simulink library "Ta_Library"  (R2019b)
settings: Solver=VariableStepAuto  StartTime=0.0  StopTime=10.0  RelTol=1e-3
undefined symbols (not defined in the file): AEBSFunctionLib, StateDelayAbortion, TargetClassification
libraries: Mylibrary x5, simulink x1
(part 2 of 3)

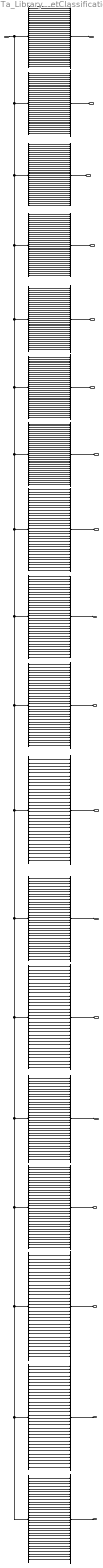
== system Ta_Library/TargetClassification ==
  Spi_input_Bus : Inport  OutDataTypeStr=Bus: Spi_input_Bus
  Bus Selector : BusSelector  OutputSignals=CAM_TGT_01A_CAN_Tgt_01_ID,CAM_TGT_02A_CAN_Tgt_02_ID,CAM_TGT_03A_CAN_Tgt_03_ID,CAM_TGT_04A_CAN_Tgt_04_ID,CAM_TGT_05A_CAN_Tgt_05_ID,CAM_TGT_06A_CAN_Tgt_06_ID,CAM_TGT_07A_CAN_Tgt_07_ID,CAM_TGT_08A_CAN_Tgt_08_ID,CAM_TGT_09A_CAN_Tgt_09_ID,CAM_TGT_10A_CAN_Tgt_10_ID,CAM_TGT_11A_CAN_Tgt_11_ID,CAM_TGT_12A_CAN_Tgt_12_ID,CAM_TGT_13A_CAN_Tgt_13_ID,CAM_TGT_14A_CAN_Tgt_14_ID,CAM_TGT_15A_CAN_Tgt_15_ID,CAM_TGT_16A_CAN_Tgt_16_ID,CAM_TGT_17A_CAN_Tgt_17_ID,CAM_TGT_18A_CAN_Tgt_18_ID,CAM_TGT_19A_CAN_Tgt_19_ID,CAM_TGT_20A_CAN_Tgt_20_ID,CAM_TGT_21A_CAN_Tgt_21_ID,CAM_TGT_22A_CAN_Tgt_22_ID,CAM_TGT_23A_CAN_Tgt_23_ID,CAM_TGT_24A_CAN_Tgt_24_ID,CAM_TGT_25A_CAN_Tgt_25_ID,CAM_TGT_26A_CAN_Tgt_26_ID,CAM_TGT_27A_CAN_Tgt_27_ID,CAM_TGT_28A_CAN_Tgt_28_ID,CAM_TGT_29A_CAN_Tgt_29_ID,CAM_TGT_30A_CAN_Tgt_30_ID,CAM_TGT_31A_CAN_Tgt_31_ID,CAM_TGT_32A_CAN_Tgt_32_ID
  Bus Selector1 : BusSelector  OutputSignals=CAM_TGT_01A_CAN_Tgt_01_Pos_Y_Quality,CAM_TGT_02A_CAN_Tgt_02_Pos_Y_Quality,CAM_TGT_03A_CAN_Tgt_03_Pos_Y_Quality,CAM_TGT_04A_CAN_Tgt_04_Pos_Y_Quality,CAM_TGT_05A_CAN_Tgt_05_Pos_Y_Quality,CAM_TGT_06A_CAN_Tgt_06_Pos_Y_Quality,CAM_TGT_07A_CAN_Tgt_07_Pos_Y_Quality,CAM_TGT_08A_CAN_Tgt_08_Pos_Y_Quality,CAM_TGT_09A_CAN_Tgt_09_Pos_Y_Quality,CAM_TGT_10A_CAN_Tgt_10_Pos_Y_Quality,CAM_TGT_11A_CAN_Tgt_11_Pos_Y_Quality,CAM_TGT_12A_CAN_Tgt_12_Pos_Y_Quality,CAM_TGT_13A_CAN_Tgt_13_Pos_Y_Quality,CAM_TGT_14A_CAN_Tgt_14_Pos_Y_Quality,CAM_TGT_15A_CAN_Tgt_15_Pos_Y_Quality,CAM_TGT_16A_CAN_Tgt_16_Pos_Y_Quality,CAM_TGT_17A_CAN_Tgt_17_Pos_Y_Quality,CAM_TGT_18A_CAN_Tgt_18_Pos_Y_Quality,CAM_TGT_19A_CAN_Tgt_19_Pos_Y_Quality,CAM_TGT_20A_CAN_Tgt_20_Pos_Y_Quality,CAM_TGT_21A_CAN_Tgt_21_Pos_Y_Quality,CAM_TGT_22A_CAN_Tgt_22_Pos_Y_Quality,CAM_TGT_23A_CAN_Tgt_23_Pos_Y_Quality,CAM_TGT_24A_CAN_Tgt_24_Pos_Y_Quality,CAM_TGT_25A_CAN_Tgt_25_Pos_Y_Quality,CAM_TGT_26A_CAN_Tgt_26_Pos_Y_Quality,CAM_TGT_27A_CAN_Tgt_27_Pos_Y_Quality,CAM_TGT_28A_CAN_Tgt_28_Pos_Y_Quality,CAM_TGT_29A_CAN_Tgt_29_Pos_Y_Quality,CAM_TGT_30A_CAN_Tgt_30_Pos_Y_Quality,CAM_TGT_31A_CAN_Tgt_31_Pos_Y_Quality,CAM_TGT_32A_CAN_Tgt_32_Pos_Y_Quality
  Bus Selector10 : BusSelector  OutputSignals=CAM_TGT_01A_CAN_Tgt_01_Pos_Y,CAM_TGT_02A_CAN_Tgt_02_Pos_Y,CAM_TGT_03A_CAN_Tgt_03_Pos_Y,CAM_TGT_04A_CAN_Tgt_04_Pos_Y,CAM_TGT_05A_CAN_Tgt_05_Pos_Y,CAM_TGT_06A_CAN_Tgt_06_Pos_Y,CAM_TGT_07A_CAN_Tgt_07_Pos_Y,CAM_TGT_08A_CAN_Tgt_08_Pos_Y,CAM_TGT_09A_CAN_Tgt_09_Pos_Y,CAM_TGT_10A_CAN_Tgt_10_Pos_Y,CAM_TGT_11A_CAN_Tgt_11_Pos_Y,CAM_TGT_12A_CAN_Tgt_12_Pos_Y,CAM_TGT_13A_CAN_Tgt_13_Pos_Y,CAM_TGT_14A_CAN_Tgt_14_Pos_Y,CAM_TGT_15A_CAN_Tgt_15_Pos_Y,CAM_TGT_16A_CAN_Tgt_16_Pos_Y,CAM_TGT_17A_CAN_Tgt_17_Pos_Y,CAM_TGT_18A_CAN_Tgt_18_Pos_Y,CAM_TGT_19A_CAN_Tgt_19_Pos_Y,CAM_TGT_20A_CAN_Tgt_20_Pos_Y,CAM_TGT_21A_CAN_Tgt_21_Pos_Y,CAM_TGT_22A_CAN_Tgt_22_Pos_Y,CAM_TGT_23A_CAN_Tgt_23_Pos_Y,CAM_TGT_24A_CAN_Tgt_24_Pos_Y,CAM_TGT_25A_CAN_Tgt_25_Pos_Y,CAM_TGT_26A_CAN_Tgt_26_Pos_Y,CAM_TGT_27A_CAN_Tgt_27_Pos_Y,CAM_TGT_28A_CAN_Tgt_28_Pos_Y,CAM_TGT_29A_CAN_Tgt_29_Pos_Y,CAM_TGT_30A_CAN_Tgt_30_Pos_Y,CAM_TGT_31A_CAN_Tgt_31_Pos_Y,CAM_TGT_32A_CAN_Tgt_32_Pos_Y
  Bus Selector11 : BusSelector  OutputSignals=CAM_TGT_01A_CAN_Tgt_01_Pos_X,CAM_TGT_02A_CAN_Tgt_02_Pos_X,CAM_TGT_03A_CAN_Tgt_03_Pos_X,CAM_TGT_04A_CAN_Tgt_04_Pos_X,CAM_TGT_05A_CAN_Tgt_05_Pos_X,CAM_TGT_06A_CAN_Tgt_06_Pos_X,CAM_TGT_07A_CAN_Tgt_07_Pos_X,CAM_TGT_08A_CAN_Tgt_08_Pos_X,CAM_TGT_09A_CAN_Tgt_09_Pos_X,CAM_TGT_10A_CAN_Tgt_10_Pos_X,CAM_TGT_11A_CAN_Tgt_11_Pos_X,CAM_TGT_12A_CAN_Tgt_12_Pos_X,CAM_TGT_13A_CAN_Tgt_13_Pos_X,CAM_TGT_14A_CAN_Tgt_14_Pos_X,CAM_TGT_15A_CAN_Tgt_15_Pos_X,CAM_TGT_16A_CAN_Tgt_16_Pos_X,CAM_TGT_17A_CAN_Tgt_17_Pos_X,CAM_TGT_18A_CAN_Tgt_18_Pos_X,CAM_TGT_19A_CAN_Tgt_19_Pos_X,CAM_TGT_20A_CAN_Tgt_20_Pos_X,CAM_TGT_21A_CAN_Tgt_21_Pos_X,CAM_TGT_22A_CAN_Tgt_22_Pos_X,CAM_TGT_23A_CAN_Tgt_23_Pos_X,CAM_TGT_24A_CAN_Tgt_24_Pos_X,CAM_TGT_25A_CAN_Tgt_25_Pos_X,CAM_TGT_26A_CAN_Tgt_26_Pos_X,CAM_TGT_27A_CAN_Tgt_27_Pos_X,CAM_TGT_28A_CAN_Tgt_28_Pos_X,CAM_TGT_29A_CAN_Tgt_29_Pos_X,CAM_TGT_30A_CAN_Tgt_30_Pos_X,CAM_TGT_31A_CAN_Tgt_31_Pos_X,CAM_TGT_32A_CAN_Tgt_32_Pos_X
  Bus Selector12 : BusSelector  OutputSignals=CAM_TGT_01B_CAN_Tgt_01_Quality,CAM_TGT_02B_CAN_Tgt_02_Quality,CAM_TGT_03B_CAN_Tgt_03_Quality,CAM_TGT_04B_CAN_Tgt_04_Quality,CAM_TGT_05B_CAN_Tgt_05_Quality,CAM_TGT_06B_CAN_Tgt_06_Quality,CAM_TGT_07B_CAN_Tgt_07_Quality,CAM_TGT_08B_CAN_Tgt_08_Quality,CAM_TGT_09B_CAN_Tgt_09_Quality,CAM_TGT_10B_CAN_Tgt_10_Quality,CAM_TGT_11B_CAN_Tgt_11_Quality,CAM_TGT_12B_CAN_Tgt_12_Quality,CAM_TGT_13B_CAN_Tgt_13_Quality,CAM_TGT_14B_CAN_Tgt_14_Quality,CAM_TGT_15B_CAN_Tgt_15_Quality,CAM_TGT_16B_CAN_Tgt_16_Quality,CAM_TGT_17B_CAN_Tgt_17_Quality,CAM_TGT_18B_CAN_Tgt_18_Quality,CAM_TGT_19B_CAN_Tgt_19_Quality,CAM_TGT_20B_CAN_Tgt_20_Quality,CAM_TGT_21B_CAN_Tgt_21_Quality,CAM_TGT_22B_CAN_Tgt_22_Quality,CAM_TGT_23B_CAN_Tgt_23_Quality,CAM_TGT_24B_CAN_Tgt_24_Quality,CAM_TGT_25B_CAN_Tgt_25_Quality,CAM_TGT_26B_CAN_Tgt_26_Quality,CAM_TGT_27B_CAN_Tgt_27_Quality,CAM_TGT_28B_CAN_Tgt_28_Quality,CAM_TGT_29B_CAN_Tgt_29_Quality,CAM_TGT_30B_CAN_Tgt_30_Quality,CAM_TGT_31B_CAN_Tgt_31_Quality,CAM_TGT_32B_CAN_Tgt_32_Quality
  Bus Selector13 : BusSelector  OutputSignals=CAM_TGT_01B_CAN_Tgt_01_Length,CAM_TGT_02B_CAN_Tgt_02_Length,CAM_TGT_03B_CAN_Tgt_03_Length,CAM_TGT_04B_CAN_Tgt_04_Length,CAM_TGT_05B_CAN_Tgt_05_Length,CAM_TGT_06B_CAN_Tgt_06_Length,CAM_TGT_07B_CAN_Tgt_07_Length,CAM_TGT_08B_CAN_Tgt_08_Length,CAM_TGT_09B_CAN_Tgt_09_Length,CAM_TGT_10B_CAN_Tgt_10_Length,CAM_TGT_11B_CAN_Tgt_11_Length,CAM_TGT_12B_CAN_Tgt_12_Length,CAM_TGT_13B_CAN_Tgt_13_Length,CAM_TGT_14B_CAN_Tgt_14_Length,CAM_TGT_15B_CAN_Tgt_15_Length,CAM_TGT_16B_CAN_Tgt_16_Length,CAM_TGT_17B_CAN_Tgt_17_Length,CAM_TGT_18B_CAN_Tgt_18_Length,CAM_TGT_19B_CAN_Tgt_19_Length,CAM_TGT_20B_CAN_Tgt_20_Length,CAM_TGT_21B_CAN_Tgt_21_Length,CAM_TGT_22B_CAN_Tgt_22_Length,CAM_TGT_23B_CAN_Tgt_23_Length,CAM_TGT_24B_CAN_Tgt_24_Length,CAM_TGT_25B_CAN_Tgt_25_Length,CAM_TGT_26B_CAN_Tgt_26_Length,CAM_TGT_27B_CAN_Tgt_27_Length,CAM_TGT_28B_CAN_Tgt_28_Length,CAM_TGT_29B_CAN_Tgt_29_Length,CAM_TGT_30B_CAN_Tgt_30_Length,CAM_TGT_31B_CAN_Tgt_31_Length,CAM_TGT_32B_CAN_Tgt_32_Length
  Bus Selector14 : BusSelector  OutputSignals=CAM_TGT_01B_CAN_Tgt_01_Time,CAM_TGT_02B_CAN_Tgt_02_Time,CAM_TGT_03B_CAN_Tgt_03_Time,CAM_TGT_04B_CAN_Tgt_04_Time,CAM_TGT_05B_CAN_Tgt_05_Time,CAM_TGT_06B_CAN_Tgt_06_Time,CAM_TGT_07B_CAN_Tgt_07_Time,CAM_TGT_08B_CAN_Tgt_08_Time,CAM_TGT_09B_CAN_Tgt_09_Time,CAM_TGT_10B_CAN_Tgt_10_Time,CAM_TGT_11B_CAN_Tgt_11_Time,CAM_TGT_12B_CAN_Tgt_12_Time,CAM_TGT_13B_CAN_Tgt_13_Time,CAM_TGT_14B_CAN_Tgt_14_Time,CAM_TGT_15B_CAN_Tgt_15_Time,CAM_TGT_16B_CAN_Tgt_16_Time,CAM_TGT_17B_CAN_Tgt_17_Time,CAM_TGT_18B_CAN_Tgt_18_Time,CAM_TGT_19B_CAN_Tgt_19_Time,CAM_TGT_20B_CAN_Tgt_20_Time,CAM_TGT_21B_CAN_Tgt_21_Time,CAM_TGT_22B_CAN_Tgt_22_Time,CAM_TGT_23B_CAN_Tgt_23_Time,CAM_TGT_24B_CAN_Tgt_24_Time,CAM_TGT_25B_CAN_Tgt_25_Time,CAM_TGT_26B_CAN_Tgt_26_Time,CAM_TGT_27B_CAN_Tgt_27_Time,CAM_TGT_28B_CAN_Tgt_28_Time,CAM_TGT_29B_CAN_Tgt_29_Time,CAM_TGT_30B_CAN_Tgt_30_Time,CAM_TGT_31B_CAN_Tgt_31_Time,CAM_TGT_32B_CAN_Tgt_32_Time
  Bus Selector15 : BusSelector  OutputSignals=CAM_TGT_01B_CAN_Tgt_01_Accel,CAM_TGT_02B_CAN_Tgt_02_Accel,CAM_TGT_03B_CAN_Tgt_03_Accel,CAM_TGT_04B_CAN_Tgt_04_Accel,CAM_TGT_05B_CAN_Tgt_05_Accel,CAM_TGT_06B_CAN_Tgt_06_Accel,CAM_TGT_07B_CAN_Tgt_07_Accel,CAM_TGT_08B_CAN_Tgt_08_Accel,CAM_TGT_09B_CAN_Tgt_09_Accel,CAM_TGT_10B_CAN_Tgt_10_Accel,CAM_TGT_11B_CAN_Tgt_11_Accel,CAM_TGT_12B_CAN_Tgt_12_Accel,CAM_TGT_13B_CAN_Tgt_13_Accel,CAM_TGT_14B_CAN_Tgt_14_Accel,CAM_TGT_15B_CAN_Tgt_15_Accel,CAM_TGT_16B_CAN_Tgt_16_Accel,CAM_TGT_17B_CAN_Tgt_17_Accel,CAM_TGT_18B_CAN_Tgt_18_Accel,CAM_TGT_19B_CAN_Tgt_19_Accel,CAM_TGT_20B_CAN_Tgt_20_Accel,CAM_TGT_21B_CAN_Tgt_21_Accel,CAM_TGT_22B_CAN_Tgt_22_Accel,CAM_TGT_23B_CAN_Tgt_23_Accel,CAM_TGT_24B_CAN_Tgt_24_Accel,CAM_TGT_25B_CAN_Tgt_25_Accel,CAM_TGT_26B_CAN_Tgt_26_Accel,CAM_TGT_27B_CAN_Tgt_27_Accel,CAM_TGT_28B_CAN_Tgt_28_Accel,CAM_TGT_29B_CAN_Tgt_29_Accel,CAM_TGT_30B_CAN_Tgt_30_Accel,CAM_TGT_31B_CAN_Tgt_31_Accel,CAM_TGT_32B_CAN_Tgt_32_Accel
  Bus Selector16 : BusSelector  OutputSignals=CAM_TGT_01B_CAN_Tgt_01_Ttc,CAM_TGT_02B_CAN_Tgt_02_Ttc,CAM_TGT_03B_CAN_Tgt_03_Ttc,CAM_TGT_04B_CAN_Tgt_04_Ttc,CAM_TGT_05B_CAN_Tgt_05_Ttc,CAM_TGT_06B_CAN_Tgt_06_Ttc,CAM_TGT_07B_CAN_Tgt_07_Ttc,CAM_TGT_08B_CAN_Tgt_08_Ttc,CAM_TGT_09B_CAN_Tgt_09_Ttc,CAM_TGT_10B_CAN_Tgt_10_Ttc,CAM_TGT_11B_CAN_Tgt_11_Ttc,CAM_TGT_12B_CAN_Tgt_12_Ttc,CAM_TGT_13B_CAN_Tgt_13_Ttc,CAM_TGT_14B_CAN_Tgt_14_Ttc,CAM_TGT_15B_CAN_Tgt_15_Ttc,CAM_TGT_16B_CAN_Tgt_16_Ttc,CAM_TGT_17B_CAN_Tgt_17_Ttc,CAM_TGT_18B_CAN_Tgt_18_Ttc,CAM_TGT_19B_CAN_Tgt_19_Ttc,CAM_TGT_20B_CAN_Tgt_20_Ttc,CAM_TGT_21B_CAN_Tgt_21_Ttc,CAM_TGT_22B_CAN_Tgt_22_Ttc,CAM_TGT_23B_CAN_Tgt_23_Ttc,CAM_TGT_24B_CAN_Tgt_24_Ttc,CAM_TGT_25B_CAN_Tgt_25_Ttc,CAM_TGT_26B_CAN_Tgt_26_Ttc,CAM_TGT_27B_CAN_Tgt_27_Ttc,CAM_TGT_28B_CAN_Tgt_28_Ttc,CAM_TGT_29B_CAN_Tgt_29_Ttc,CAM_TGT_30B_CAN_Tgt_30_Ttc,CAM_TGT_31B_CAN_Tgt_31_Ttc,CAM_TGT_32B_CAN_Tgt_32_Ttc
  Bus Selector17 : BusSelector  OutputSignals=CAM_TGT_01B_CAN_Tgt_01_Width,CAM_TGT_02B_CAN_Tgt_02_Width,CAM_TGT_03B_CAN_Tgt_03_Width,CAM_TGT_04B_CAN_Tgt_04_Width,CAM_TGT_05B_CAN_Tgt_05_Width,CAM_TGT_06B_CAN_Tgt_06_Width,CAM_TGT_07B_CAN_Tgt_07_Width,CAM_TGT_08B_CAN_Tgt_08_Width,CAM_TGT_09B_CAN_Tgt_09_Width,CAM_TGT_10B_CAN_Tgt_10_Width,CAM_TGT_11B_CAN_Tgt_11_Width,CAM_TGT_12B_CAN_Tgt_12_Width,CAM_TGT_13B_CAN_Tgt_13_Width,CAM_TGT_14B_CAN_Tgt_14_Width,CAM_TGT_15B_CAN_Tgt_15_Width,CAM_TGT_16B_CAN_Tgt_16_Width,CAM_TGT_17B_CAN_Tgt_17_Width,CAM_TGT_18B_CAN_Tgt_18_Width,CAM_TGT_19B_CAN_Tgt_19_Width,CAM_TGT_20B_CAN_Tgt_20_Width,CAM_TGT_21B_CAN_Tgt_21_Width,CAM_TGT_22B_CAN_Tgt_22_Width,CAM_TGT_23B_CAN_Tgt_23_Width,CAM_TGT_24B_CAN_Tgt_24_Width,CAM_TGT_25B_CAN_Tgt_25_Width,CAM_TGT_26B_CAN_Tgt_26_Width,CAM_TGT_27B_CAN_Tgt_27_Width,CAM_TGT_28B_CAN_Tgt_28_Width,CAM_TGT_29B_CAN_Tgt_29_Width,CAM_TGT_30B_CAN_Tgt_30_Width,CAM_TGT_31B_CAN_Tgt_31_Width,CAM_TGT_32B_CAN_Tgt_32_Width
  Bus Selector2 : BusSelector  OutputSignals=CAM_TGT_01A_CAN_Tgt_01_Type,CAM_TGT_02A_CAN_Tgt_02_Type,CAM_TGT_03A_CAN_Tgt_03_Type,CAM_TGT_04A_CAN_Tgt_04_Type,CAM_TGT_05A_CAN_Tgt_05_Type,CAM_TGT_06A_CAN_Tgt_06_Type,CAM_TGT_07A_CAN_Tgt_07_Type,CAM_TGT_08A_CAN_Tgt_08_Type,CAM_TGT_09A_CAN_Tgt_09_Type,CAM_TGT_10A_CAN_Tgt_10_Type,CAM_TGT_11A_CAN_Tgt_11_Type,CAM_TGT_12A_CAN_Tgt_12_Type,CAM_TGT_13A_CAN_Tgt_13_Type,CAM_TGT_14A_CAN_Tgt_14_Type,CAM_TGT_15A_CAN_Tgt_15_Type,CAM_TGT_16A_CAN_Tgt_16_Type,CAM_TGT_17A_CAN_Tgt_17_Type,CAM_TGT_18A_CAN_Tgt_18_Type,CAM_TGT_19A_CAN_Tgt_19_Type,CAM_TGT_20A_CAN_Tgt_20_Type,CAM_TGT_21A_CAN_Tgt_21_Type,CAM_TGT_22A_CAN_Tgt_22_Type,CAM_TGT_23A_CAN_Tgt_23_Type,CAM_TGT_24A_CAN_Tgt_24_Type,CAM_TGT_25A_CAN_Tgt_25_Type,CAM_TGT_26A_CAN_Tgt_26_Type,CAM_TGT_27A_CAN_Tgt_27_Type,CAM_TGT_28A_CAN_Tgt_28_Type,CAM_TGT_29A_CAN_Tgt_29_Type,CAM_TGT_30A_CAN_Tgt_30_Type,CAM_TGT_31A_CAN_Tgt_31_Type,CAM_TGT_32A_CAN_Tgt_32_Type
  Bus Selector3 : BusSelector  OutputSignals=CAM_TGT_01A_CAN_Tgt_01_Spd_X_Quality,CAM_TGT_02A_CAN_Tgt_02_Spd_X_Quality,CAM_TGT_03A_CAN_Tgt_03_Spd_X_Quality,CAM_TGT_04A_CAN_Tgt_04_Spd_X_Quality,CAM_TGT_05A_CAN_Tgt_05_Spd_X_Quality,CAM_TGT_06A_CAN_Tgt_06_Spd_X_Quality,CAM_TGT_07A_CAN_Tgt_07_Spd_X_Quality,CAM_TGT_08A_CAN_Tgt_08_Spd_X_Quality,CAM_TGT_09A_CAN_Tgt_09_Spd_X_Quality,CAM_TGT_10A_CAN_Tgt_10_Spd_X_Quality,CAM_TGT_11A_CAN_Tgt_11_Spd_X_Quality,CAM_TGT_12A_CAN_Tgt_12_Spd_X_Quality,CAM_TGT_13A_CAN_Tgt_13_Spd_X_Quality,CAM_TGT_14A_CAN_Tgt_14_Spd_X_Quality,CAM_TGT_15A_CAN_Tgt_15_Spd_X_Quality,CAM_TGT_16A_CAN_Tgt_16_Spd_X_Quality,CAM_TGT_17A_CAN_Tgt_17_Spd_X_Quality,CAM_TGT_18A_CAN_Tgt_18_Spd_X_Quality,CAM_TGT_19A_CAN_Tgt_19_Spd_X_Quality,CAM_TGT_20A_CAN_Tgt_20_Spd_X_Quality,CAM_TGT_21A_CAN_Tgt_21_Spd_X_Quality,CAM_TGT_22A_CAN_Tgt_22_Spd_X_Quality,CAM_TGT_23A_CAN_Tgt_23_Spd_X_Quality,CAM_TGT_24A_CAN_Tgt_24_Spd_X_Quality,CAM_TGT_25A_CAN_Tgt_25_Spd_X_Quality,CAM_TGT_26A_CAN_Tgt_26_Spd_X_Quality,CAM_TGT_27A_CAN_Tgt_27_Spd_X_Quality,CAM_TGT_28A_CAN_Tgt_28_Spd_X_Quality,CAM_TGT_29A_CAN_Tgt_29_Spd_X_Quality,CAM_TGT_30A_CAN_Tgt_30_Spd_X_Quality,CAM_TGT_31A_CAN_Tgt_31_Spd_X_Quality,CAM_TGT_32A_CAN_Tgt_32_Spd_X_Quality
  Bus Selector4 : BusSelector  OutputSignals=CAM_TGT_01A_CAN_Tgt_01_Pos_X_Quality,CAM_TGT_02A_CAN_Tgt_02_Pos_X_Quality,CAM_TGT_03A_CAN_Tgt_03_Pos_X_Quality,CAM_TGT_04A_CAN_Tgt_04_Pos_X_Quality,CAM_TGT_05A_CAN_Tgt_05_Pos_X_Quality,CAM_TGT_06A_CAN_Tgt_06_Pos_X_Quality,CAM_TGT_07A_CAN_Tgt_07_Pos_X_Quality,CAM_TGT_08A_CAN_Tgt_08_Pos_X_Quality,CAM_TGT_09A_CAN_Tgt_09_Pos_X_Quality,CAM_TGT_10A_CAN_Tgt_10_Pos_X_Quality,CAM_TGT_11A_CAN_Tgt_11_Pos_X_Quality,CAM_TGT_12A_CAN_Tgt_12_Pos_X_Quality,CAM_TGT_13A_CAN_Tgt_13_Pos_X_Quality,CAM_TGT_14A_CAN_Tgt_14_Pos_X_Quality,CAM_TGT_15A_CAN_Tgt_15_Pos_X_Quality,CAM_TGT_16A_CAN_Tgt_16_Pos_X_Quality,CAM_TGT_17A_CAN_Tgt_17_Pos_X_Quality,CAM_TGT_18A_CAN_Tgt_18_Pos_X_Quality,CAM_TGT_19A_CAN_Tgt_19_Pos_X_Quality,CAM_TGT_20A_CAN_Tgt_20_Pos_X_Quality,CAM_TGT_21A_CAN_Tgt_21_Pos_X_Quality,CAM_TGT_22A_CAN_Tgt_22_Pos_X_Quality,CAM_TGT_23A_CAN_Tgt_23_Pos_X_Quality,CAM_TGT_24A_CAN_Tgt_24_Pos_X_Quality,CAM_TGT_25A_CAN_Tgt_25_Pos_X_Quality,CAM_TGT_26A_CAN_Tgt_26_Pos_X_Quality,CAM_TGT_27A_CAN_Tgt_27_Pos_X_Quality,CAM_TGT_28A_CAN_Tgt_28_Pos_X_Quality,CAM_TGT_29A_CAN_Tgt_29_Pos_X_Quality,CAM_TGT_30A_CAN_Tgt_30_Pos_X_Quality,CAM_TGT_31A_CAN_Tgt_31_Pos_X_Quality,CAM_TGT_32A_CAN_Tgt_32_Pos_X_Quality
  Bus Selector5 : BusSelector  OutputSignals=CAM_TGT_01A_CAN_Tgt_01_Behavior,CAM_TGT_02A_CAN_Tgt_02_Behavior,CAM_TGT_03A_CAN_Tgt_03_Behavior,CAM_TGT_04A_CAN_Tgt_04_Behavior,CAM_TGT_05A_CAN_Tgt_05_Behavior,CAM_TGT_06A_CAN_Tgt_06_Behavior,CAM_TGT_07A_CAN_Tgt_07_Behavior,CAM_TGT_08A_CAN_Tgt_08_Behavior,CAM_TGT_09A_CAN_Tgt_09_Behavior,CAM_TGT_10A_CAN_Tgt_10_Behavior,CAM_TGT_11A_CAN_Tgt_11_Behavior,CAM_TGT_12A_CAN_Tgt_12_Behavior,CAM_TGT_13A_CAN_Tgt_13_Behavior,CAM_TGT_14A_CAN_Tgt_14_Behavior,CAM_TGT_15A_CAN_Tgt_15_Behavior,CAM_TGT_16A_CAN_Tgt_16_Behavior,CAM_TGT_17A_CAN_Tgt_17_Behavior,CAM_TGT_18A_CAN_Tgt_18_Behavior,CAM_TGT_19A_CAN_Tgt_19_Behavior,CAM_TGT_20A_CAN_Tgt_20_Behavior,CAM_TGT_21A_CAN_Tgt_21_Behavior,CAM_TGT_22A_CAN_Tgt_22_Behavior,CAM_TGT_23A_CAN_Tgt_23_Behavior,CAM_TGT_24A_CAN_Tgt_24_Behavior,CAM_TGT_25A_CAN_Tgt_25_Behavior,CAM_TGT_26A_CAN_Tgt_26_Behavior,CAM_TGT_27A_CAN_Tgt_27_Behavior,CAM_TGT_28A_CAN_Tgt_28_Behavior,CAM_TGT_29A_CAN_Tgt_29_Behavior,CAM_TGT_30A_CAN_Tgt_30_Behavior,CAM_TGT_31A_CAN_Tgt_31_Behavior,CAM_TGT_32A_CAN_Tgt_32_Behavior
  Bus Selector6 : BusSelector  OutputSignals=CAM_TGT_01A_CAN_Tgt_01_Stat,CAM_TGT_02A_CAN_Tgt_02_Stat,CAM_TGT_03A_CAN_Tgt_03_Stat,CAM_TGT_04A_CAN_Tgt_04_Stat,CAM_TGT_05A_CAN_Tgt_05_Stat,CAM_TGT_06A_CAN_Tgt_06_Stat,CAM_TGT_07A_CAN_Tgt_07_Stat,CAM_TGT_08A_CAN_Tgt_08_Stat,CAM_TGT_09A_CAN_Tgt_09_Stat,CAM_TGT_10A_CAN_Tgt_10_Stat,CAM_TGT_11A_CAN_Tgt_11_Stat,CAM_TGT_12A_CAN_Tgt_12_Stat,CAM_TGT_13A_CAN_Tgt_13_Stat,CAM_TGT_14A_CAN_Tgt_14_Stat,CAM_TGT_15A_CAN_Tgt_15_Stat,CAM_TGT_16A_CAN_Tgt_16_Stat,CAM_TGT_17A_CAN_Tgt_17_Stat,CAM_TGT_18A_CAN_Tgt_18_Stat,CAM_TGT_19A_CAN_Tgt_19_Stat,CAM_TGT_20A_CAN_Tgt_20_Stat,CAM_TGT_21A_CAN_Tgt_21_Stat,CAM_TGT_22A_CAN_Tgt_22_Stat,CAM_TGT_23A_CAN_Tgt_23_Stat,CAM_TGT_24A_CAN_Tgt_24_Stat,CAM_TGT_25A_CAN_Tgt_25_Stat,CAM_TGT_26A_CAN_Tgt_26_Stat,CAM_TGT_27A_CAN_Tgt_27_Stat,CAM_TGT_28A_CAN_Tgt_28_Stat,CAM_TGT_29A_CAN_Tgt_29_Stat,CAM_TGT_30A_CAN_Tgt_30_Stat,CAM_TGT_31A_CAN_Tgt_31_Stat,CAM_TGT_32A_CAN_Tgt_32_Stat
  Bus Selector7 : BusSelector  OutputSignals=CAM_TGT_01A_CAN_Tgt_01_Spd_Y_Quality,CAM_TGT_02A_CAN_Tgt_02_Spd_Y_Quality,CAM_TGT_03A_CAN_Tgt_03_Spd_Y_Quality,CAM_TGT_04A_CAN_Tgt_04_Spd_Y_Quality,CAM_TGT_05A_CAN_Tgt_05_Spd_Y_Quality,CAM_TGT_06A_CAN_Tgt_06_Spd_Y_Quality,CAM_TGT_07A_CAN_Tgt_07_Spd_Y_Quality,CAM_TGT_08A_CAN_Tgt_08_Spd_Y_Quality,CAM_TGT_09A_CAN_Tgt_09_Spd_Y_Quality,CAM_TGT_10A_CAN_Tgt_10_Spd_Y_Quality,CAM_TGT_11A_CAN_Tgt_11_Spd_Y_Quality,CAM_TGT_12A_CAN_Tgt_12_Spd_Y_Quality,CAM_TGT_13A_CAN_Tgt_13_Spd_Y_Quality,CAM_TGT_14A_CAN_Tgt_14_Spd_Y_Quality,CAM_TGT_15A_CAN_Tgt_15_Spd_Y_Quality,CAM_TGT_16A_CAN_Tgt_16_Spd_Y_Quality,CAM_TGT_17A_CAN_Tgt_17_Spd_Y_Quality,CAM_TGT_18A_CAN_Tgt_18_Spd_Y_Quality,CAM_TGT_19A_CAN_Tgt_19_Spd_Y_Quality,CAM_TGT_20A_CAN_Tgt_20_Spd_Y_Quality,CAM_TGT_21A_CAN_Tgt_21_Spd_Y_Quality,CAM_TGT_22A_CAN_Tgt_22_Spd_Y_Quality,CAM_TGT_23A_CAN_Tgt_23_Spd_Y_Quality,CAM_TGT_24A_CAN_Tgt_24_Spd_Y_Quality,CAM_TGT_25A_CAN_Tgt_25_Spd_Y_Quality,CAM_TGT_26A_CAN_Tgt_26_Spd_Y_Quality,CAM_TGT_27A_CAN_Tgt_27_Spd_Y_Quality,CAM_TGT_28A_CAN_Tgt_28_Spd_Y_Quality,CAM_TGT_29A_CAN_Tgt_29_Spd_Y_Quality,CAM_TGT_30A_CAN_Tgt_30_Spd_Y_Quality,CAM_TGT_31A_CAN_Tgt_31_Spd_Y_Quality,CAM_TGT_32A_CAN_Tgt_32_Spd_Y_Quality
  Bus Selector8 : BusSelector  OutputSignals=CAM_TGT_01A_CAN_Tgt_01_Spd_X,CAM_TGT_02A_CAN_Tgt_02_Spd_X,CAM_TGT_03A_CAN_Tgt_03_Spd_X,CAM_TGT_04A_CAN_Tgt_04_Spd_X,CAM_TGT_05A_CAN_Tgt_05_Spd_X,CAM_TGT_06A_CAN_Tgt_06_Spd_X,CAM_TGT_07A_CAN_Tgt_07_Spd_X,CAM_TGT_08A_CAN_Tgt_08_Spd_X,CAM_TGT_09A_CAN_Tgt_09_Spd_X,CAM_TGT_10A_CAN_Tgt_10_Spd_X,CAM_TGT_11A_CAN_Tgt_11_Spd_X,CAM_TGT_12A_CAN_Tgt_12_Spd_X,CAM_TGT_13A_CAN_Tgt_13_Spd_X,CAM_TGT_14A_CAN_Tgt_14_Spd_X,CAM_TGT_15A_CAN_Tgt_15_Spd_X,CAM_TGT_16A_CAN_Tgt_16_Spd_X,CAM_TGT_17A_CAN_Tgt_17_Spd_X,CAM_TGT_18A_CAN_Tgt_18_Spd_X,CAM_TGT_19A_CAN_Tgt_19_Spd_X,CAM_TGT_20A_CAN_Tgt_20_Spd_X,CAM_TGT_21A_CAN_Tgt_21_Spd_X,CAM_TGT_22A_CAN_Tgt_22_Spd_X,CAM_TGT_23A_CAN_Tgt_23_Spd_X,CAM_TGT_24A_CAN_Tgt_24_Spd_X,CAM_TGT_25A_CAN_Tgt_25_Spd_X,CAM_TGT_26A_CAN_Tgt_26_Spd_X,CAM_TGT_27A_CAN_Tgt_27_Spd_X,CAM_TGT_28A_CAN_Tgt_28_Spd_X,CAM_TGT_29A_CAN_Tgt_29_Spd_X,CAM_TGT_30A_CAN_Tgt_30_Spd_X,CAM_TGT_31A_CAN_Tgt_31_Spd_X,CAM_TGT_32A_CAN_Tgt_32_Spd_X
  Bus Selector9 : BusSelector  OutputSignals=CAM_TGT_01A_CAN_Tgt_01_Spd_Y,CAM_TGT_02A_CAN_Tgt_02_Spd_Y,CAM_TGT_03A_CAN_Tgt_03_Spd_Y,CAM_TGT_04A_CAN_Tgt_04_Spd_Y,CAM_TGT_05A_CAN_Tgt_05_Spd_Y,CAM_TGT_06A_CAN_Tgt_06_Spd_Y,CAM_TGT_07A_CAN_Tgt_07_Spd_Y,CAM_TGT_08A_CAN_Tgt_08_Spd_Y,CAM_TGT_09A_CAN_Tgt_09_Spd_Y,CAM_TGT_10A_CAN_Tgt_10_Spd_Y,CAM_TGT_11A_CAN_Tgt_11_Spd_Y,CAM_TGT_12A_CAN_Tgt_12_Spd_Y,CAM_TGT_13A_CAN_Tgt_13_Spd_Y,CAM_TGT_14A_CAN_Tgt_14_Spd_Y,CAM_TGT_15A_CAN_Tgt_15_Spd_Y,CAM_TGT_16A_CAN_Tgt_16_Spd_Y,CAM_TGT_17A_CAN_Tgt_17_Spd_Y,CAM_TGT_18A_CAN_Tgt_18_Spd_Y,CAM_TGT_19A_CAN_Tgt_19_Spd_Y,CAM_TGT_20A_CAN_Tgt_20_Spd_Y,CAM_TGT_21A_CAN_Tgt_21_Spd_Y,CAM_TGT_22A_CAN_Tgt_22_Spd_Y,CAM_TGT_23A_CAN_Tgt_23_Spd_Y,CAM_TGT_24A_CAN_Tgt_24_Spd_Y,CAM_TGT_25A_CAN_Tgt_25_Spd_Y,CAM_TGT_26A_CAN_Tgt_26_Spd_Y,CAM_TGT_27A_CAN_Tgt_27_Spd_Y,CAM_TGT_28A_CAN_Tgt_28_Spd_Y,CAM_TGT_29A_CAN_Tgt_29_Spd_Y,CAM_TGT_30A_CAN_Tgt_30_Spd_Y,CAM_TGT_31A_CAN_Tgt_31_Spd_Y,CAM_TGT_32A_CAN_Tgt_32_Spd_Y
  Mux{,1..17} (18 alike) : Mux  Inputs=32
  ID : Outport
  Pos_Y_Quality : Outport  Port=2
  Type : Outport  Port=3
  Spd_X_Quality : Outport  Port=4
  Pos_X_Quality : Outport  Port=5
  Behavior : Outport  Port=6
  Stat : Outport  Port=7
  Spd_Y_Quality : Outport  Port=8
  Spd_X : Outport  Port=9
  Spd_Y : Outport  Port=10
  Pos_Y : Outport  Port=11
  Pos_X : Outport  Port=12
  Quality : Outport  Port=13
  Length : Outport  Port=14
  Time : Outport  Port=15
  Accel : Outport  Port=16
  Ttc : Outport  Port=17
  Width : Outport  Port=18
  wires:
  Bus Selector/1 -> Mux/1  "<CAM_TGT_01A_CAN_Tgt_01_ID>"
  Bus Selector12/27 -> Mux12/27  "<CAM_TGT_27B_CAN_Tgt_27_Quality>"
  Bus Selector12/20 -> Mux12/20  "<CAM_TGT_20B_CAN_Tgt_20_Quality>"
  Mux7/1 -> Spd_Y_Quality/1
  Bus Selector16/4 -> Mux16/4  "<CAM_TGT_04B_CAN_Tgt_04_Ttc>"
  Bus Selector10/17 -> Mux10/17  "<CAM_TGT_17A_CAN_Tgt_17_Pos_Y>"
  Bus Selector15/4 -> Mux15/4  "<CAM_TGT_04B_CAN_Tgt_04_Accel>"
  Bus Selector3/8 -> Mux3/8  "<CAM_TGT_08A_CAN_Tgt_08_Spd_X_Quality>"
  Bus Selector6/17 -> Mux6/17  "<CAM_TGT_17A_CAN_Tgt_17_Stat>"
  Bus Selector15/18 -> Mux15/18  "<CAM_TGT_18B_CAN_Tgt_18_Accel>"
  Bus Selector6/3 -> Mux6/3  "<CAM_TGT_03A_CAN_Tgt_03_Stat>"
  Bus Selector5/7 -> Mux5/7  "<CAM_TGT_07A_CAN_Tgt_07_Behavior>"
  Bus Selector7/32 -> Mux7/32  "<CAM_TGT_32A_CAN_Tgt_32_Spd_Y_Quality>"
  Bus Selector1/3 -> Mux1/3  "<CAM_TGT_03A_CAN_Tgt_03_Pos_Y_Quality>"
  Bus Selector12/22 -> Mux12/22  "<CAM_TGT_22B_CAN_Tgt_22_Quality>"
  Bus Selector10/18 -> Mux10/18  "<CAM_TGT_18A_CAN_Tgt_18_Pos_Y>"
  Bus Selector12/30 -> Mux12/30  "<CAM_TGT_30B_CAN_Tgt_30_Quality>"
  Bus Selector14/2 -> Mux14/2  "<CAM_TGT_02B_CAN_Tgt_02_Time>"
  Bus Selector9/29 -> Mux9/29  "<CAM_TGT_29A_CAN_Tgt_29_Spd_Y>"
  Bus Selector12/16 -> Mux12/16  "<CAM_TGT_16B_CAN_Tgt_16_Quality>"
  Bus Selector12/1 -> Mux12/1  "<CAM_TGT_01B_CAN_Tgt_01_Quality>"
  Bus Selector4/12 -> Mux4/12  "<CAM_TGT_12A_CAN_Tgt_12_Pos_X_Quality>"
  Bus Selector12/19 -> Mux12/19  "<CAM_TGT_19B_CAN_Tgt_19_Quality>"
  Bus Selector17/32 -> Mux17/32  "<CAM_TGT_32B_CAN_Tgt_32_Width>"
  Bus Selector16/2 -> Mux16/2  "<CAM_TGT_02B_CAN_Tgt_02_Ttc>"
  Bus Selector5/20 -> Mux5/20  "<CAM_TGT_20A_CAN_Tgt_20_Behavior>"
  Bus Selector11/31 -> Mux11/31  "<CAM_TGT_31A_CAN_Tgt_31_Pos_X>"
  Bus Selector14/15 -> Mux14/15  "<CAM_TGT_15B_CAN_Tgt_15_Time>"
  Bus Selector16/30 -> Mux16/30  "<CAM_TGT_30B_CAN_Tgt_30_Ttc>"
  Bus Selector12/28 -> Mux12/28  "<CAM_TGT_28B_CAN_Tgt_28_Quality>"
  Bus Selector12/25 -> Mux12/25  "<CAM_TGT_25B_CAN_Tgt_25_Quality>"
  Mux4/1 -> Pos_X_Quality/1
  Bus Selector6/32 -> Mux6/32  "<CAM_TGT_32A_CAN_Tgt_32_Stat>"
  Bus Selector15/15 -> Mux15/15  "<CAM_TGT_15B_CAN_Tgt_15_Accel>"
  Bus Selector17/10 -> Mux17/10  "<CAM_TGT_10B_CAN_Tgt_10_Width>"
  Bus Selector17/9 -> Mux17/9  "<CAM_TGT_09B_CAN_Tgt_09_Width>"
  Bus Selector15/5 -> Mux15/5  "<CAM_TGT_05B_CAN_Tgt_05_Accel>"
  Bus Selector8/7 -> Mux8/7  "<CAM_TGT_07A_CAN_Tgt_07_Spd_X>"
  Mux11/1 -> Pos_X/1
  Bus Selector1/25 -> Mux1/25  "<CAM_TGT_25A_CAN_Tgt_25_Pos_Y_Quality>"
  Bus Selector14/31 -> Mux14/31  "<CAM_TGT_31B_CAN_Tgt_31_Time>"
  Bus Selector5/30 -> Mux5/30  "<CAM_TGT_30A_CAN_Tgt_30_Behavior>"
  Bus Selector7/20 -> Mux7/20  "<CAM_TGT_20A_CAN_Tgt_20_Spd_Y_Quality>"
  Mux17/1 -> Width/1
  Bus Selector13/21 -> Mux13/21  "<CAM_TGT_21B_CAN_Tgt_21_Length>"
  Bus Selector5/31 -> Mux5/31  "<CAM_TGT_31A_CAN_Tgt_31_Behavior>"
  Bus Selector13/2 -> Mux13/2  "<CAM_TGT_02B_CAN_Tgt_02_Length>"
  Bus Selector12/21 -> Mux12/21  "<CAM_TGT_21B_CAN_Tgt_21_Quality>"
  Bus Selector15/13 -> Mux15/13  "<CAM_TGT_13B_CAN_Tgt_13_Accel>"
  Bus Selector10/19 -> Mux10/19  "<CAM_TGT_19A_CAN_Tgt_19_Pos_Y>"
  Bus Selector/29 -> Mux/29  "<CAM_TGT_29A_CAN_Tgt_29_ID>"
  Bus Selector8/28 -> Mux8/28  "<CAM_TGT_28A_CAN_Tgt_28_Spd_X>"
  Bus Selector1/13 -> Mux1/13  "<CAM_TGT_13A_CAN_Tgt_13_Pos_Y_Quality>"
  Bus Selector1/2 -> Mux1/2  "<CAM_TGT_02A_CAN_Tgt_02_Pos_Y_Quality>"
  Bus Selector4/26 -> Mux4/26  "<CAM_TGT_26A_CAN_Tgt_26_Pos_X_Quality>"
  Bus Selector3/32 -> Mux3/32  "<CAM_TGT_32A_CAN_Tgt_32_Spd_X_Quality>"
  Bus Selector12/18 -> Mux12/18  "<CAM_TGT_18B_CAN_Tgt_18_Quality>"
  Bus Selector16/22 -> Mux16/22  "<CAM_TGT_22B_CAN_Tgt_22_Ttc>"
  Bus Selector10/16 -> Mux10/16  "<CAM_TGT_16A_CAN_Tgt_16_Pos_Y>"
  Bus Selector12/24 -> Mux12/24  "<CAM_TGT_24B_CAN_Tgt_24_Quality>"
  Bus Selector10/26 -> Mux10/26  "<CAM_TGT_26A_CAN_Tgt_26_Pos_Y>"
  Bus Selector6/26 -> Mux6/26  "<CAM_TGT_26A_CAN_Tgt_26_Stat>"
  Bus Selector/21 -> Mux/21  "<CAM_TGT_21A_CAN_Tgt_21_ID>"
  Bus Selector12/26 -> Mux12/26  "<CAM_TGT_26B_CAN_Tgt_26_Quality>"
  Bus Selector17/14 -> Mux17/14  "<CAM_TGT_14B_CAN_Tgt_14_Width>"
  Bus Selector12/32 -> Mux12/32  "<CAM_TGT_32B_CAN_Tgt_32_Quality>"
  Bus Selector1/29 -> Mux1/29  "<CAM_TGT_29A_CAN_Tgt_29_Pos_Y_Quality>"
  Bus Selector9/28 -> Mux9/28  "<CAM_TGT_28A_CAN_Tgt_28_Spd_Y>"
  Bus Selector11/28 -> Mux11/28  "<CAM_TGT_28A_CAN_Tgt_28_Pos_X>"
  Bus Selector10/7 -> Mux10/7  "<CAM_TGT_07A_CAN_Tgt_07_Pos_Y>"
  Bus Selector9/13 -> Mux9/13  "<CAM_TGT_13A_CAN_Tgt_13_Spd_Y>"
  Bus Selector16/5 -> Mux16/5  "<CAM_TGT_05B_CAN_Tgt_05_Ttc>"
  Bus Selector11/16 -> Mux11/16  "<CAM_TGT_16A_CAN_Tgt_16_Pos_X>"
  Bus Selector14/11 -> Mux14/11  "<CAM_TGT_11B_CAN_Tgt_11_Time>"
  Spi_input_Bus/1 -> Bus Selector17/1, Bus Selector16/1, Bus Selector15/1, Bus Selector14/1, Bus Selector13/1, Bus Selector12/1, Bus Selector11/1, Bus Selector10/1, Bus Selector9/1, Bus Selector8/1, Bus Selector7/1, Bus Selector6/1, Bus Selector5/1, Bus Selector4/1, Bus Selector3/1, Bus Selector2/1, Bus Selector1/1, Bus Selector/1
  Bus Selector12/29 -> Mux12/29  "<CAM_TGT_29B_CAN_Tgt_29_Quality>"
  Bus Selector6/30 -> Mux6/30  "<CAM_TGT_30A_CAN_Tgt_30_Stat>"
  Bus Selector8/18 -> Mux8/18  "<CAM_TGT_18A_CAN_Tgt_18_Spd_X>"
  Bus Selector/2 -> Mux/2  "<CAM_TGT_02A_CAN_Tgt_02_ID>"
  Bus Selector1/26 -> Mux1/26  "<CAM_TGT_26A_CAN_Tgt_26_Pos_Y_Quality>"
  Bus Selector6/21 -> Mux6/21  "<CAM_TGT_21A_CAN_Tgt_21_Stat>"
  Bus Selector2/28 -> Mux2/28  "<CAM_TGT_28A_CAN_Tgt_28_Type>"
  Bus Selector12/23 -> Mux12/23  "<CAM_TGT_23B_CAN_Tgt_23_Quality>"
  Bus Selector3/9 -> Mux3/9  "<CAM_TGT_09A_CAN_Tgt_09_Spd_X_Quality>"
  Bus Selector12/11 -> Mux12/11  "<CAM_TGT_11B_CAN_Tgt_11_Quality>"
  Bus Selector9/8 -> Mux9/8  "<CAM_TGT_08A_CAN_Tgt_08_Spd_Y>"
  Bus Selector11/22 -> Mux11/22  "<CAM_TGT_22A_CAN_Tgt_22_Pos_X>"
  Bus Selector16/11 -> Mux16/11  "<CAM_TGT_11B_CAN_Tgt_11_Ttc>"
  Bus Selector12/7 -> Mux12/7  "<CAM_TGT_07B_CAN_Tgt_07_Quality>"
  Bus Selector/22 -> Mux/22  "<CAM_TGT_22A_CAN_Tgt_22_ID>"
  Bus Selector16/20 -> Mux16/20  "<CAM_TGT_20B_CAN_Tgt_20_Ttc>"
  Bus Selector8/21 -> Mux8/21  "<CAM_TGT_21A_CAN_Tgt_21_Spd_X>"
  Bus Selector4/32 -> Mux4/32  "<CAM_TGT_32A_CAN_Tgt_32_Pos_X_Quality>"
  Bus Selector8/9 -> Mux8/9  "<CAM_TGT_09A_CAN_Tgt_09_Spd_X>"
  Bus Selector13/13 -> Mux13/13  "<CAM_TGT_13B_CAN_Tgt_13_Length>"
  Bus Selector2/4 -> Mux2/4  "<CAM_TGT_04A_CAN_Tgt_04_Type>"
  Bus Selector3/20 -> Mux3/20  "<CAM_TGT_20A_CAN_Tgt_20_Spd_X_Quality>"
  Bus Selector9/25 -> Mux9/25  "<CAM_TGT_25A_CAN_Tgt_25_Spd_Y>"
  Bus Selector4/13 -> Mux4/13  "<CAM_TGT_13A_CAN_Tgt_13_Pos_X_Quality>"
  Bus Selector10/32 -> Mux10/32  "<CAM_TGT_32A_CAN_Tgt_32_Pos_Y>"
  Bus Selector10/15 -> Mux10/15  "<CAM_TGT_15A_CAN_Tgt_15_Pos_Y>"
  Bus Selector9/5 -> Mux9/5  "<CAM_TGT_05A_CAN_Tgt_05_Spd_Y>"
  Bus Selector16/23 -> Mux16/23  "<CAM_TGT_23B_CAN_Tgt_23_Ttc>"
  Bus Selector12/31 -> Mux12/31  "<CAM_TGT_31B_CAN_Tgt_31_Quality>"
  Bus Selector1/9 -> Mux1/9  "<CAM_TGT_09A_CAN_Tgt_09_Pos_Y_Quality>"
  Bus Selector9/24 -> Mux9/24  "<CAM_TGT_24A_CAN_Tgt_24_Spd_Y>"
  Bus Selector12/8 -> Mux12/8  "<CAM_TGT_08B_CAN_Tgt_08_Quality>"
  Bus Selector10/23 -> Mux10/23  "<CAM_TGT_23A_CAN_Tgt_23_Pos_Y>"
  Bus Selector14/29 -> Mux14/29  "<CAM_TGT_29B_CAN_Tgt_29_Time>"
  Bus Selector13/31 -> Mux13/31  "<CAM_TGT_31B_CAN_Tgt_31_Length>"
  Bus Selector17/3 -> Mux17/3  "<CAM_TGT_03B_CAN_Tgt_03_Width>"
  Bus Selector8/20 -> Mux8/20  "<CAM_TGT_20A_CAN_Tgt_20_Spd_X>"
  Bus Selector12/6 -> Mux12/6  "<CAM_TGT_06B_CAN_Tgt_06_Quality>"
  Bus Selector5/3 -> Mux5/3  "<CAM_TGT_03A_CAN_Tgt_03_Behavior>"
  Bus Selector6/23 -> Mux6/23  "<CAM_TGT_23A_CAN_Tgt_23_Stat>"
  Bus Selector7/12 -> Mux7/12  "<CAM_TGT_12A_CAN_Tgt_12_Spd_Y_Quality>"
  Bus Selector9/19 -> Mux9/19  "<CAM_TGT_19A_CAN_Tgt_19_Spd_Y>"
  Bus Selector6/4 -> Mux6/4  "<CAM_TGT_04A_CAN_Tgt_04_Stat>"
  Bus Selector16/26 -> Mux16/26  "<CAM_TGT_26B_CAN_Tgt_26_Ttc>"
  Bus Selector6/7 -> Mux6/7  "<CAM_TGT_07A_CAN_Tgt_07_Stat>"
  Bus Selector7/7 -> Mux7/7  "<CAM_TGT_07A_CAN_Tgt_07_Spd_Y_Quality>"
  Bus Selector9/20 -> Mux9/20  "<CAM_TGT_20A_CAN_Tgt_20_Spd_Y>"
  Bus Selector12/4 -> Mux12/4  "<CAM_TGT_04B_CAN_Tgt_04_Quality>"
  Bus Selector2/13 -> Mux2/13  "<CAM_TGT_13A_CAN_Tgt_13_Type>"
  Bus Selector16/28 -> Mux16/28  "<CAM_TGT_28B_CAN_Tgt_28_Ttc>"
  Bus Selector8/23 -> Mux8/23  "<CAM_TGT_23A_CAN_Tgt_23_Spd_X>"
  Bus Selector13/12 -> Mux13/12  "<CAM_TGT_12B_CAN_Tgt_12_Length>"
  Bus Selector17/6 -> Mux17/6  "<CAM_TGT_06B_CAN_Tgt_06_Width>"
  Bus Selector8/25 -> Mux8/25  "<CAM_TGT_25A_CAN_Tgt_25_Spd_X>"
  Bus Selector9/31 -> Mux9/31  "<CAM_TGT_31A_CAN_Tgt_31_Spd_Y>"
  Bus Selector14/13 -> Mux14/13  "<CAM_TGT_13B_CAN_Tgt_13_Time>"
  Bus Selector12/3 -> Mux12/3  "<CAM_TGT_03B_CAN_Tgt_03_Quality>"
  Bus Selector12/2 -> Mux12/2  "<CAM_TGT_02B_CAN_Tgt_02_Quality>"
  Bus Selector8/24 -> Mux8/24  "<CAM_TGT_24A_CAN_Tgt_24_Spd_X>"
  Bus Selector12/5 -> Mux12/5  "<CAM_TGT_05B_CAN_Tgt_05_Quality>"
  Bus Selector14/19 -> Mux14/19  "<CAM_TGT_19B_CAN_Tgt_19_Time>"
  Bus Selector5/13 -> Mux5/13  "<CAM_TGT_13A_CAN_Tgt_13_Behavior>"
  Bus Selector11/13 -> Mux11/13  "<CAM_TGT_13A_CAN_Tgt_13_Pos_X>"
  Bus Selector12/12 -> Mux12/12  "<CAM_TGT_12B_CAN_Tgt_12_Quality>"
  Bus Selector/10 -> Mux/10  "<CAM_TGT_10A_CAN_Tgt_10_ID>"
  Bus Selector12/9 -> Mux12/9  "<CAM_TGT_09B_CAN_Tgt_09_Quality>"
  Bus Selector2/1 -> Mux2/1  "<CAM_TGT_01A_CAN_Tgt_01_Type>"
  Bus Selector1/4 -> Mux1/4  "<CAM_TGT_04A_CAN_Tgt_04_Pos_Y_Quality>"
  Bus Selector2/20 -> Mux2/20  "<CAM_TGT_20A_CAN_Tgt_20_Type>"
  Mux10/1 -> Pos_Y/1
  Bus Selector13/28 -> Mux13/28  "<CAM_TGT_28B_CAN_Tgt_28_Length>"
  Bus Selector13/25 -> Mux13/25  "<CAM_TGT_25B_CAN_Tgt_25_Length>"
  Bus Selector11/18 -> Mux11/18  "<CAM_TGT_18A_CAN_Tgt_18_Pos_X>"
  Bus Selector1/18 -> Mux1/18  "<CAM_TGT_18A_CAN_Tgt_18_Pos_Y_Quality>"
  Bus Selector5/24 -> Mux5/24  "<CAM_TGT_24A_CAN_Tgt_24_Behavior>"
  Bus Selector11/27 -> Mux11/27  "<CAM_TGT_27A_CAN_Tgt_27_Pos_X>"
  Bus Selector11/10 -> Mux11/10  "<CAM_TGT_10A_CAN_Tgt_10_Pos_X>"
  Bus Selector7/21 -> Mux7/21  "<CAM_TGT_21A_CAN_Tgt_21_Spd_Y_Quality>"
  Bus Selector12/10 -> Mux12/10  "<CAM_TGT_10B_CAN_Tgt_10_Quality>"
  Bus Selector16/27 -> Mux16/27  "<CAM_TGT_27B_CAN_Tgt_27_Ttc>"
  Bus Selector17/4 -> Mux17/4  "<CAM_TGT_04B_CAN_Tgt_04_Width>"
  Bus Selector11/9 -> Mux11/9  "<CAM_TGT_09A_CAN_Tgt_09_Pos_X>"
  Bus Selector4/29 -> Mux4/29  "<CAM_TGT_29A_CAN_Tgt_29_Pos_X_Quality>"
  Bus Selector14/22 -> Mux14/22  "<CAM_TGT_22B_CAN_Tgt_22_Time>"
  Bus Selector/7 -> Mux/7  "<CAM_TGT_07A_CAN_Tgt_07_ID>"
  Bus Selector12/15 -> Mux12/15  "<CAM_TGT_15B_CAN_Tgt_15_Quality>"
  Bus Selector12/14 -> Mux12/14  "<CAM_TGT_14B_CAN_Tgt_14_Quality>"
  Bus Selector12/17 -> Mux12/17  "<CAM_TGT_17B_CAN_Tgt_17_Quality>"
  Bus Selector12/13 -> Mux12/13  "<CAM_TGT_13B_CAN_Tgt_13_Quality>"
  Bus Selector2/32 -> Mux2/32  "<CAM_TGT_32A_CAN_Tgt_32_Type>"
  Bus Selector10/30 -> Mux10/30  "<CAM_TGT_30A_CAN_Tgt_30_Pos_Y>"
  Bus Selector1/1 -> Mux1/1  "<CAM_TGT_01A_CAN_Tgt_01_Pos_Y_Quality>"
  Bus Selector10/1 -> Mux10/1  "<CAM_TGT_01A_CAN_Tgt_01_Pos_Y>"
  Bus Selector11/19 -> Mux11/19  "<CAM_TGT_19A_CAN_Tgt_19_Pos_X>"
  Bus Selector11/25 -> Mux11/25  "<CAM_TGT_25A_CAN_Tgt_25_Pos_X>"
  Bus Selector1/21 -> Mux1/21  "<CAM_TGT_21A_CAN_Tgt_21_Pos_Y_Quality>"
  Bus Selector4/25 -> Mux4/25  "<CAM_TGT_25A_CAN_Tgt_25_Pos_X_Quality>"
  Bus Selector6/6 -> Mux6/6  "<CAM_TGT_06A_CAN_Tgt_06_Stat>"
  Bus Selector6/19 -> Mux6/19  "<CAM_TGT_19A_CAN_Tgt_19_Stat>"
  Bus Selector/8 -> Mux/8  "<CAM_TGT_08A_CAN_Tgt_08_ID>"
  Bus Selector2/9 -> Mux2/9  "<CAM_TGT_09A_CAN_Tgt_09_Type>"
  Bus Selector13/29 -> Mux13/29  "<CAM_TGT_29B_CAN_Tgt_29_Length>"
  Bus Selector10/5 -> Mux10/5  "<CAM_TGT_05A_CAN_Tgt_05_Pos_Y>"
  Bus Selector11/1 -> Mux11/1  "<CAM_TGT_01A_CAN_Tgt_01_Pos_X>"
  Bus Selector2/17 -> Mux2/17  "<CAM_TGT_17A_CAN_Tgt_17_Type>"
  Bus Selector1/10 -> Mux1/10  "<CAM_TGT_10A_CAN_Tgt_10_Pos_Y_Quality>"
  Bus Selector7/3 -> Mux7/3  "<CAM_TGT_03A_CAN_Tgt_03_Spd_Y_Quality>"
  Bus Selector9/6 -> Mux9/6  "<CAM_TGT_06A_CAN_Tgt_06_Spd_Y>"
  Bus Selector15/20 -> Mux15/20  "<CAM_TGT_20B_CAN_Tgt_20_Accel>"
  Bus Selector1/5 -> Mux1/5  "<CAM_TGT_05A_CAN_Tgt_05_Pos_Y_Quality>"
  Bus Selector10/3 -> Mux10/3  "<CAM_TGT_03A_CAN_Tgt_03_Pos_Y>"
  Bus Selector1/11 -> Mux1/11  "<CAM_TGT_11A_CAN_Tgt_11_Pos_Y_Quality>"
  Bus Selector1/30 -> Mux1/30  "<CAM_TGT_30A_CAN_Tgt_30_Pos_Y_Quality>"
  Bus Selector2/29 -> Mux2/29  "<CAM_TGT_29A_CAN_Tgt_29_Type>"
  Bus Selector1/7 -> Mux1/7  "<CAM_TGT_07A_CAN_Tgt_07_Pos_Y_Quality>"
  Bus Selector1/32 -> Mux1/32  "<CAM_TGT_32A_CAN_Tgt_32_Pos_Y_Quality>"
  Bus Selector3/13 -> Mux3/13  "<CAM_TGT_13A_CAN_Tgt_13_Spd_X_Quality>"
  Bus Selector5/1 -> Mux5/1  "<CAM_TGT_01A_CAN_Tgt_01_Behavior>"
  Bus Selector4/22 -> Mux4/22  "<CAM_TGT_22A_CAN_Tgt_22_Pos_X_Quality>"
  Bus Selector1/17 -> Mux1/17  "<CAM_TGT_17A_CAN_Tgt_17_Pos_Y_Quality>"
  Bus Selector1/6 -> Mux1/6  "<CAM_TGT_06A_CAN_Tgt_06_Pos_Y_Quality>"
  Bus Selector11/21 -> Mux11/21  "<CAM_TGT_21A_CAN_Tgt_21_Pos_X>"
  Bus Selector13/30 -> Mux13/30  "<CAM_TGT_30B_CAN_Tgt_30_Length>"
  Bus Selector4/15 -> Mux4/15  "<CAM_TGT_15A_CAN_Tgt_15_Pos_X_Quality>"
  Bus Selector17/7 -> Mux17/7  "<CAM_TGT_07B_CAN_Tgt_07_Width>"
  Bus Selector1/8 -> Mux1/8  "<CAM_TGT_08A_CAN_Tgt_08_Pos_Y_Quality>"
  Bus Selector17/2 -> Mux17/2  "<CAM_TGT_02B_CAN_Tgt_02_Width>"
  Mux3/1 -> Spd_X_Quality/1
  Bus Selector4/31 -> Mux4/31  "<CAM_TGT_31A_CAN_Tgt_31_Pos_X_Quality>"
  Bus Selector1/12 -> Mux1/12  "<CAM_TGT_12A_CAN_Tgt_12_Pos_Y_Quality>"
  Bus Selector1/14 -> Mux1/14  "<CAM_TGT_14A_CAN_Tgt_14_Pos_Y_Quality>"
  Bus Selector3/29 -> Mux3/29  "<CAM_TGT_29A_CAN_Tgt_29_Spd_X_Quality>"
  Bus Selector14/9 -> Mux14/9  "<CAM_TGT_09B_CAN_Tgt_09_Time>"
  Bus Selector5/23 -> Mux5/23  "<CAM_TGT_23A_CAN_Tgt_23_Behavior>"
  Bus Selector1/16 -> Mux1/16  "<CAM_TGT_16A_CAN_Tgt_16_Pos_Y_Quality>"
  Bus Selector1/15 -> Mux1/15  "<CAM_TGT_15A_CAN_Tgt_15_Pos_Y_Quality>"
  Bus Selector11/11 -> Mux11/11  "<CAM_TGT_11A_CAN_Tgt_11_Pos_X>"
  Bus Selector14/16 -> Mux14/16  "<CAM_TGT_16B_CAN_Tgt_16_Time>"
  Bus Selector1/20 -> Mux1/20  "<CAM_TGT_20A_CAN_Tgt_20_Pos_Y_Quality>"
  Bus Selector13/27 -> Mux13/27  "<CAM_TGT_27B_CAN_Tgt_27_Length>"
  Bus Selector16/25 -> Mux16/25  "<CAM_TGT_25B_CAN_Tgt_25_Ttc>"
  Mux12/1 -> Quality/1
  Bus Selector1/22 -> Mux1/22  "<CAM_TGT_22A_CAN_Tgt_22_Pos_Y_Quality>"
  Bus Selector7/22 -> Mux7/22  "<CAM_TGT_22A_CAN_Tgt_22_Spd_Y_Quality>"
  Bus Selector9/32 -> Mux9/32  "<CAM_TGT_32A_CAN_Tgt_32_Spd_Y>"
  Bus Selector11/26 -> Mux11/26  "<CAM_TGT_26A_CAN_Tgt_26_Pos_X>"
  Bus Selector7/30 -> Mux7/30  "<CAM_TGT_30A_CAN_Tgt_30_Spd_Y_Quality>"
  Bus Selector5/28 -> Mux5/28  "<CAM_TGT_28A_CAN_Tgt_28_Behavior>"
  Bus Selector1/23 -> Mux1/23  "<CAM_TGT_23A_CAN_Tgt_23_Pos_Y_Quality>"
  Bus Selector7/10 -> Mux7/10  "<CAM_TGT_10A_CAN_Tgt_10_Spd_Y_Quality>"
  Mux5/1 -> Behavior/1
  Bus Selector1/27 -> Mux1/27  "<CAM_TGT_27A_CAN_Tgt_27_Pos_Y_Quality>"
  Bus Selector6/25 -> Mux6/25  "<CAM_TGT_25A_CAN_Tgt_25_Stat>"
  Bus Selector13/22 -> Mux13/22  "<CAM_TGT_22B_CAN_Tgt_22_Length>"
  Bus Selector1/19 -> Mux1/19  "<CAM_TGT_19A_CAN_Tgt_19_Pos_Y_Quality>"
  Bus Selector4/4 -> Mux4/4  "<CAM_TGT_04A_CAN_Tgt_04_Pos_X_Quality>"
  Bus Selector14/7 -> Mux14/7  "<CAM_TGT_07B_CAN_Tgt_07_Time>"
  Bus Selector1/28 -> Mux1/28  "<CAM_TGT_28A_CAN_Tgt_28_Pos_Y_Quality>"
  Bus Selector7/18 -> Mux7/18  "<CAM_TGT_18A_CAN_Tgt_18_Spd_Y_Quality>"
  Bus Selector7/13 -> Mux7/13  "<CAM_TGT_13A_CAN_Tgt_13_Spd_Y_Quality>"
  Bus Selector14/24 -> Mux14/24  "<CAM_TGT_24B_CAN_Tgt_24_Time>"
  Bus Selector14/6 -> Mux14/6  "<CAM_TGT_06B_CAN_Tgt_06_Time>"
  Bus Selector17/26 -> Mux17/26  "<CAM_TGT_26B_CAN_Tgt_26_Width>"
  Bus Selector1/24 -> Mux1/24  "<CAM_TGT_24A_CAN_Tgt_24_Pos_Y_Quality>"
  Bus Selector15/32 -> Mux15/32  "<CAM_TGT_32B_CAN_Tgt_32_Accel>"
  Bus Selector/25 -> Mux/25  "<CAM_TGT_25A_CAN_Tgt_25_ID>"
  Bus Selector5/21 -> Mux5/21  "<CAM_TGT_21A_CAN_Tgt_21_Behavior>"
  Bus Selector2/31 -> Mux2/31  "<CAM_TGT_31A_CAN_Tgt_31_Type>"
  Bus Selector17/5 -> Mux17/5  "<CAM_TGT_05B_CAN_Tgt_05_Width>"
  Bus Selector13/11 -> Mux13/11  "<CAM_TGT_11B_CAN_Tgt_11_Length>"
  Bus Selector13/14 -> Mux13/14  "<CAM_TGT_14B_CAN_Tgt_14_Length>"
  Bus Selector1/31 -> Mux1/31  "<CAM_TGT_31A_CAN_Tgt_31_Pos_Y_Quality>"
  Bus Selector7/17 -> Mux7/17  "<CAM_TGT_17A_CAN_Tgt_17_Spd_Y_Quality>"
  Bus Selector2/3 -> Mux2/3  "<CAM_TGT_03A_CAN_Tgt_03_Type>"
  Bus Selector2/16 -> Mux2/16  "<CAM_TGT_16A_CAN_Tgt_16_Type>"
  Bus Selector9/30 -> Mux9/30  "<CAM_TGT_30A_CAN_Tgt_30_Spd_Y>"
  Bus Selector2/15 -> Mux2/15  "<CAM_TGT_15A_CAN_Tgt_15_Type>"
  Bus Selector/32 -> Mux/32  "<CAM_TGT_32A_CAN_Tgt_32_ID>"
  Bus Selector5/6 -> Mux5/6  "<CAM_TGT_06A_CAN_Tgt_06_Behavior>"
  Bus Selector4/21 -> Mux4/21  "<CAM_TGT_21A_CAN_Tgt_21_Pos_X_Quality>"
  Bus Selector14/3 -> Mux14/3  "<CAM_TGT_03B_CAN_Tgt_03_Time>"
  Bus Selector/15 -> Mux/15  "<CAM_TGT_15A_CAN_Tgt_15_ID>"
  Bus Selector2/18 -> Mux2/18  "<CAM_TGT_18A_CAN_Tgt_18_Type>"
  Bus Selector6/27 -> Mux6/27  "<CAM_TGT_27A_CAN_Tgt_27_Stat>"
  Bus Selector/4 -> Mux/4  "<CAM_TGT_04A_CAN_Tgt_04_ID>"
  Bus Selector3/22 -> Mux3/22  "<CAM_TGT_22A_CAN_Tgt_22_Spd_X_Quality>"
  Bus Selector3/18 -> Mux3/18  "<CAM_TGT_18A_CAN_Tgt_18_Spd_X_Quality>"
  Bus Selector2/14 -> Mux2/14  "<CAM_TGT_14A_CAN_Tgt_14_Type>"
  Bus Selector6/9 -> Mux6/9  "<CAM_TGT_09A_CAN_Tgt_09_Stat>"
  Bus Selector2/19 -> Mux2/19  "<CAM_TGT_19A_CAN_Tgt_19_Type>"
  Bus Selector4/9 -> Mux4/9  "<CAM_TGT_09A_CAN_Tgt_09_Pos_X_Quality>"
  Bus Selector4/20 -> Mux4/20  "<CAM_TGT_20A_CAN_Tgt_20_Pos_X_Quality>"
  Bus Selector15/6 -> Mux15/6  "<CAM_TGT_06B_CAN_Tgt_06_Accel>"
  Bus Selector2/26 -> Mux2/26  "<CAM_TGT_26A_CAN_Tgt_26_Type>"
  Bus Selector2/25 -> Mux2/25  "<CAM_TGT_25A_CAN_Tgt_25_Type>"
  Bus Selector6/5 -> Mux6/5  "<CAM_TGT_05A_CAN_Tgt_05_Stat>"
  Bus Selector7/28 -> Mux7/28  "<CAM_TGT_28A_CAN_Tgt_28_Spd_Y_Quality>"
  Bus Selector2/23 -> Mux2/23  "<CAM_TGT_23A_CAN_Tgt_23_Type>"
  Bus Selector2/21 -> Mux2/21  "<CAM_TGT_21A_CAN_Tgt_21_Type>"
  Bus Selector2/22 -> Mux2/22  "<CAM_TGT_22A_CAN_Tgt_22_Type>"
  Bus Selector16/14 -> Mux16/14  "<CAM_TGT_14B_CAN_Tgt_14_Ttc>"
  Bus Selector7/31 -> Mux7/31  "<CAM_TGT_31A_CAN_Tgt_31_Spd_Y_Quality>"
  Bus Selector5/29 -> Mux5/29  "<CAM_TGT_29A_CAN_Tgt_29_Behavior>"
  Bus Selector2/24 -> Mux2/24  "<CAM_TGT_24A_CAN_Tgt_24_Type>"
  Bus Selector10/24 -> Mux10/24  "<CAM_TGT_24A_CAN_Tgt_24_Pos_Y>"
  Bus Selector5/32 -> Mux5/32  "<CAM_TGT_32A_CAN_Tgt_32_Behavior>"
  Bus Selector2/27 -> Mux2/27  "<CAM_TGT_27A_CAN_Tgt_27_Type>"
  Bus Selector7/4 -> Mux7/4  "<CAM_TGT_04A_CAN_Tgt_04_Spd_Y_Quality>"
  Bus Selector14/23 -> Mux14/23  "<CAM_TGT_23B_CAN_Tgt_23_Time>"
  Bus Selector7/6 -> Mux7/6  "<CAM_TGT_06A_CAN_Tgt_06_Spd_Y_Quality>"
  Bus Selector16/31 -> Mux16/31  "<CAM_TGT_31B_CAN_Tgt_31_Ttc>"
  Bus Selector2/30 -> Mux2/30  "<CAM_TGT_30A_CAN_Tgt_30_Type>"
  Bus Selector17/18 -> Mux17/18  "<CAM_TGT_18B_CAN_Tgt_18_Width>"
  Mux2/1 -> Type/1
  Bus Selector14/5 -> Mux14/5  "<CAM_TGT_05B_CAN_Tgt_05_Time>"
  Bus Selector2/7 -> Mux2/7  "<CAM_TGT_07A_CAN_Tgt_07_Type>"
  Bus Selector9/11 -> Mux9/11  "<CAM_TGT_11A_CAN_Tgt_11_Spd_Y>"
  Bus Selector/14 -> Mux/14  "<CAM_TGT_14A_CAN_Tgt_14_ID>"
  Mux6/1 -> Stat/1
  Bus Selector16/29 -> Mux16/29  "<CAM_TGT_29B_CAN_Tgt_29_Ttc>"
  Bus Selector5/19 -> Mux5/19  "<CAM_TGT_19A_CAN_Tgt_19_Behavior>"
  Bus Selector14/4 -> Mux14/4  "<CAM_TGT_04B_CAN_Tgt_04_Time>"
  Bus Selector6/20 -> Mux6/20  "<CAM_TGT_20A_CAN_Tgt_20_Stat>"
  Bus Selector14/8 -> Mux14/8  "<CAM_TGT_08B_CAN_Tgt_08_Time>"
  Bus Selector14/10 -> Mux14/10  "<CAM_TGT_10B_CAN_Tgt_10_Time>"
  Bus Selector5/5 -> Mux5/5  "<CAM_TGT_05A_CAN_Tgt_05_Behavior>"
  Bus Selector14/12 -> Mux14/12  "<CAM_TGT_12B_CAN_Tgt_12_Time>"
  Mux9/1 -> Spd_Y/1
  Bus Selector14/14 -> Mux14/14  "<CAM_TGT_14B_CAN_Tgt_14_Time>"
  Bus Selector17/22 -> Mux17/22  "<CAM_TGT_22B_CAN_Tgt_22_Width>"
  Mux16/1 -> Ttc/1
  Bus Selector8/11 -> Mux8/11  "<CAM_TGT_11A_CAN_Tgt_11_Spd_X>"
  Bus Selector4/18 -> Mux4/18  "<CAM_TGT_18A_CAN_Tgt_18_Pos_X_Quality>"
  Bus Selector/9 -> Mux/9  "<CAM_TGT_09A_CAN_Tgt_09_ID>"
  Bus Selector3/24 -> Mux3/24  "<CAM_TGT_24A_CAN_Tgt_24_Spd_X_Quality>"
  Bus Selector14/18 -> Mux14/18  "<CAM_TGT_18B_CAN_Tgt_18_Time>"
  Bus Selector11/5 -> Mux11/5  "<CAM_TGT_05A_CAN_Tgt_05_Pos_X>"
  Bus Selector5/26 -> Mux5/26  "<CAM_TGT_26A_CAN_Tgt_26_Behavior>"
  Bus Selector14/17 -> Mux14/17  "<CAM_TGT_17B_CAN_Tgt_17_Time>"
  Bus Selector/5 -> Mux/5  "<CAM_TGT_05A_CAN_Tgt_05_ID>"
  Bus Selector4/6 -> Mux4/6  "<CAM_TGT_06A_CAN_Tgt_06_Pos_X_Quality>"
  Bus Selector7/27 -> Mux7/27  "<CAM_TGT_27A_CAN_Tgt_27_Spd_Y_Quality>"
  Bus Selector2/11 -> Mux2/11  "<CAM_TGT_11A_CAN_Tgt_11_Type>"
  Bus Selector14/21 -> Mux14/21  "<CAM_TGT_21B_CAN_Tgt_21_Time>"
  Bus Selector14/20 -> Mux14/20  "<CAM_TGT_20B_CAN_Tgt_20_Time>"
  Bus Selector14/25 -> Mux14/25  "<CAM_TGT_25B_CAN_Tgt_25_Time>"
  Bus Selector/13 -> Mux/13  "<CAM_TGT_13A_CAN_Tgt_13_ID>"
  Bus Selector15/25 -> Mux15/25  "<CAM_TGT_25B_CAN_Tgt_25_Accel>"
  Bus Selector3/4 -> Mux3/4  "<CAM_TGT_04A_CAN_Tgt_04_Spd_X_Quality>"
  Bus Selector17/17 -> Mux17/17  "<CAM_TGT_17B_CAN_Tgt_17_Width>"
  Bus Selector6/8 -> Mux6/8  "<CAM_TGT_08A_CAN_Tgt_08_Stat>"
  Bus Selector5/12 -> Mux5/12  "<CAM_TGT_12A_CAN_Tgt_12_Behavior>"
  Bus Selector15/28 -> Mux15/28  "<CAM_TGT_28B_CAN_Tgt_28_Accel>"
  Mux15/1 -> Accel/1
  Bus Selector14/27 -> Mux14/27  "<CAM_TGT_27B_CAN_Tgt_27_Time>"
  Bus Selector/6 -> Mux/6  "<CAM_TGT_06A_CAN_Tgt_06_ID>"
  Bus Selector14/26 -> Mux14/26  "<CAM_TGT_26B_CAN_Tgt_26_Time>"
  Bus Selector13/8 -> Mux13/8  "<CAM_TGT_08B_CAN_Tgt_08_Length>"
  Bus Selector10/29 -> Mux10/29  "<CAM_TGT_29A_CAN_Tgt_29_Pos_Y>"
  Bus Selector4/16 -> Mux4/16  "<CAM_TGT_16A_CAN_Tgt_16_Pos_X_Quality>"
  Bus Selector14/28 -> Mux14/28  "<CAM_TGT_28B_CAN_Tgt_28_Time>"
  Bus Selector14/30 -> Mux14/30  "<CAM_TGT_30B_CAN_Tgt_30_Time>"
  Bus Selector14/32 -> Mux14/32  "<CAM_TGT_32B_CAN_Tgt_32_Time>"
  Bus Selector2/2 -> Mux2/2  "<CAM_TGT_02A_CAN_Tgt_02_Type>"
  Bus Selector14/1 -> Mux14/1  "<CAM_TGT_01B_CAN_Tgt_01_Time>"
  Bus Selector8/10 -> Mux8/10  "<CAM_TGT_10A_CAN_Tgt_10_Spd_X>"
  Bus Selector6/16 -> Mux6/16  "<CAM_TGT_16A_CAN_Tgt_16_Stat>"
  Bus Selector6/12 -> Mux6/12  "<CAM_TGT_12A_CAN_Tgt_12_Stat>"
  Bus Selector3/16 -> Mux3/16  "<CAM_TGT_16A_CAN_Tgt_16_Spd_X_Quality>"
  Bus Selector7/14 -> Mux7/14  "<CAM_TGT_14A_CAN_Tgt_14_Spd_Y_Quality>"
  Mux14/1 -> Time/1
  Bus Selector5/22 -> Mux5/22  "<CAM_TGT_22A_CAN_Tgt_22_Behavior>"
  Bus Selector7/25 -> Mux7/25  "<CAM_TGT_25A_CAN_Tgt_25_Spd_Y_Quality>"
  Bus Selector/31 -> Mux/31  "<CAM_TGT_31A_CAN_Tgt_31_ID>"
  Bus Selector9/18 -> Mux9/18  "<CAM_TGT_18A_CAN_Tgt_18_Spd_Y>"
  Bus Selector2/5 -> Mux2/5  "<CAM_TGT_05A_CAN_Tgt_05_Type>"
  Bus Selector4/17 -> Mux4/17  "<CAM_TGT_17A_CAN_Tgt_17_Pos_X_Quality>"
  Bus Selector5/27 -> Mux5/27  "<CAM_TGT_27A_CAN_Tgt_27_Behavior>"
  Bus Selector13/4 -> Mux13/4  "<CAM_TGT_04B_CAN_Tgt_04_Length>"
  Bus Selector5/4 -> Mux5/4  "<CAM_TGT_04A_CAN_Tgt_04_Behavior>"
  Bus Selector2/6 -> Mux2/6  "<CAM_TGT_06A_CAN_Tgt_06_Type>"
  Bus Selector16/19 -> Mux16/19  "<CAM_TGT_19B_CAN_Tgt_19_Ttc>"
  Bus Selector4/2 -> Mux4/2  "<CAM_TGT_02A_CAN_Tgt_02_Pos_X_Quality>"
  Bus Selector15/22 -> Mux15/22  "<CAM_TGT_22B_CAN_Tgt_22_Accel>"
  Bus Selector10/14 -> Mux10/14  "<CAM_TGT_14A_CAN_Tgt_14_Pos_Y>"
  Bus Selector2/10 -> Mux2/10  "<CAM_TGT_10A_CAN_Tgt_10_Type>"
  Bus Selector3/15 -> Mux3/15  "<CAM_TGT_15A_CAN_Tgt_15_Spd_X_Quality>"
  Bus Selector8/13 -> Mux8/13  "<CAM_TGT_13A_CAN_Tgt_13_Spd_X>"
  Bus Selector2/8 -> Mux2/8  "<CAM_TGT_08A_CAN_Tgt_08_Type>"
  Bus Selector2/12 -> Mux2/12  "<CAM_TGT_12A_CAN_Tgt_12_Type>"
  Bus Selector10/8 -> Mux10/8  "<CAM_TGT_08A_CAN_Tgt_08_Pos_Y>"
  Bus Selector17/1 -> Mux17/1  "<CAM_TGT_01B_CAN_Tgt_01_Width>"
  Bus Selector8/6 -> Mux8/6  "<CAM_TGT_06A_CAN_Tgt_06_Spd_X>"
  Bus Selector9/14 -> Mux9/14  "<CAM_TGT_14A_CAN_Tgt_14_Spd_Y>"
  Bus Selector17/8 -> Mux17/8  "<CAM_TGT_08B_CAN_Tgt_08_Width>"
  Bus Selector/12 -> Mux/12  "<CAM_TGT_12A_CAN_Tgt_12_ID>"
  Bus Selector5/25 -> Mux5/25  "<CAM_TGT_25A_CAN_Tgt_25_Behavior>"
  Bus Selector10/9 -> Mux10/9  "<CAM_TGT_09A_CAN_Tgt_09_Pos_Y>"
  Bus Selector17/12 -> Mux17/12  "<CAM_TGT_12B_CAN_Tgt_12_Width>"
  Bus Selector17/11 -> Mux17/11  "<CAM_TGT_11B_CAN_Tgt_11_Width>"
  Bus Selector15/3 -> Mux15/3  "<CAM_TGT_03B_CAN_Tgt_03_Accel>"
  Bus Selector17/16 -> Mux17/16  "<CAM_TGT_16B_CAN_Tgt_16_Width>"
  Bus Selector11/20 -> Mux11/20  "<CAM_TGT_20A_CAN_Tgt_20_Pos_X>"
  Bus Selector7/23 -> Mux7/23  "<CAM_TGT_23A_CAN_Tgt_23_Spd_Y_Quality>"
  Bus Selector17/15 -> Mux17/15  "<CAM_TGT_15B_CAN_Tgt_15_Width>"
  Bus Selector5/15 -> Mux5/15  "<CAM_TGT_15A_CAN_Tgt_15_Behavior>"
  Bus Selector17/13 -> Mux17/13  "<CAM_TGT_13B_CAN_Tgt_13_Width>"
  Bus Selector16/3 -> Mux16/3  "<CAM_TGT_03B_CAN_Tgt_03_Ttc>"
  Bus Selector8/1 -> Mux8/1  "<CAM_TGT_01A_CAN_Tgt_01_Spd_X>"
  Bus Selector10/4 -> Mux10/4  "<CAM_TGT_04A_CAN_Tgt_04_Pos_Y>"
  Bus Selector17/19 -> Mux17/19  "<CAM_TGT_19B_CAN_Tgt_19_Width>"
  Bus Selector7/15 -> Mux7/15  "<CAM_TGT_15A_CAN_Tgt_15_Spd_Y_Quality>"
  Bus Selector17/20 -> Mux17/20  "<CAM_TGT_20B_CAN_Tgt_20_Width>"
  Bus Selector17/21 -> Mux17/21  "<CAM_TGT_21B_CAN_Tgt_21_Width>"
  Bus Selector17/27 -> Mux17/27  "<CAM_TGT_27B_CAN_Tgt_27_Width>"
  Bus Selector3/12 -> Mux3/12  "<CAM_TGT_12A_CAN_Tgt_12_Spd_X_Quality>"
  Bus Selector8/30 -> Mux8/30  "<CAM_TGT_30A_CAN_Tgt_30_Spd_X>"
  Bus Selector17/25 -> Mux17/25  "<CAM_TGT_25B_CAN_Tgt_25_Width>"
  Bus Selector4/30 -> Mux4/30  "<CAM_TGT_30A_CAN_Tgt_30_Pos_X_Quality>"
  Bus Selector17/23 -> Mux17/23  "<CAM_TGT_23B_CAN_Tgt_23_Width>"
  Bus Selector17/24 -> Mux17/24  "<CAM_TGT_24B_CAN_Tgt_24_Width>"
  Bus Selector/18 -> Mux/18  "<CAM_TGT_18A_CAN_Tgt_18_ID>"
  Bus Selector15/12 -> Mux15/12  "<CAM_TGT_12B_CAN_Tgt_12_Accel>"
  Bus Selector16/32 -> Mux16/32  "<CAM_TGT_32B_CAN_Tgt_32_Ttc>"
  Bus Selector17/30 -> Mux17/30  "<CAM_TGT_30B_CAN_Tgt_30_Width>"
  Bus Selector17/31 -> Mux17/31  "<CAM_TGT_31B_CAN_Tgt_31_Width>"
  Bus Selector17/29 -> Mux17/29  "<CAM_TGT_29B_CAN_Tgt_29_Width>"
  Bus Selector17/28 -> Mux17/28  "<CAM_TGT_28B_CAN_Tgt_28_Width>"
  Bus Selector8/15 -> Mux8/15  "<CAM_TGT_15A_CAN_Tgt_15_Spd_X>"
  Bus Selector9/2 -> Mux9/2  "<CAM_TGT_02A_CAN_Tgt_02_Spd_Y>"
  Bus Selector9/4 -> Mux9/4  "<CAM_TGT_04A_CAN_Tgt_04_Spd_Y>"
  Bus Selector9/3 -> Mux9/3  "<CAM_TGT_03A_CAN_Tgt_03_Spd_Y>"
  Bus Selector9/9 -> Mux9/9  "<CAM_TGT_09A_CAN_Tgt_09_Spd_Y>"
  Bus Selector4/1 -> Mux4/1  "<CAM_TGT_01A_CAN_Tgt_01_Pos_X_Quality>"
  Bus Selector9/7 -> Mux9/7  "<CAM_TGT_07A_CAN_Tgt_07_Spd_Y>"
  Bus Selector9/10 -> Mux9/10  "<CAM_TGT_10A_CAN_Tgt_10_Spd_Y>"
  Bus Selector15/8 -> Mux15/8  "<CAM_TGT_08B_CAN_Tgt_08_Accel>"
  Bus Selector/26 -> Mux/26  "<CAM_TGT_26A_CAN_Tgt_26_ID>"
  Bus Selector10/10 -> Mux10/10  "<CAM_TGT_10A_CAN_Tgt_10_Pos_Y>"
  Bus Selector3/23 -> Mux3/23  "<CAM_TGT_23A_CAN_Tgt_23_Spd_X_Quality>"
  Bus Selector9/12 -> Mux9/12  "<CAM_TGT_12A_CAN_Tgt_12_Spd_Y>"
  Bus Selector16/9 -> Mux16/9  "<CAM_TGT_09B_CAN_Tgt_09_Ttc>"
  Bus Selector9/15 -> Mux9/15  "<CAM_TGT_15A_CAN_Tgt_15_Spd_Y>"
  Bus Selector4/8 -> Mux4/8  "<CAM_TGT_08A_CAN_Tgt_08_Pos_X_Quality>"
  Bus Selector6/10 -> Mux6/10  "<CAM_TGT_10A_CAN_Tgt_10_Stat>"
  Bus Selector9/17 -> Mux9/17  "<CAM_TGT_17A_CAN_Tgt_17_Spd_Y>"
  Bus Selector16/18 -> Mux16/18  "<CAM_TGT_18B_CAN_Tgt_18_Ttc>"
  Bus Selector13/32 -> Mux13/32  "<CAM_TGT_32B_CAN_Tgt_32_Length>"
  Bus Selector9/16 -> Mux9/16  "<CAM_TGT_16A_CAN_Tgt_16_Spd_Y>"
  Bus Selector5/8 -> Mux5/8  "<CAM_TGT_08A_CAN_Tgt_08_Behavior>"
  Bus Selector9/23 -> Mux9/23  "<CAM_TGT_23A_CAN_Tgt_23_Spd_Y>"
  Bus Selector16/21 -> Mux16/21  "<CAM_TGT_21B_CAN_Tgt_21_Ttc>"
  Bus Selector9/22 -> Mux9/22  "<CAM_TGT_22A_CAN_Tgt_22_Spd_Y>"
  Bus Selector9/21 -> Mux9/21  "<CAM_TGT_21A_CAN_Tgt_21_Spd_Y>"
  Bus Selector5/10 -> Mux5/10  "<CAM_TGT_10A_CAN_Tgt_10_Behavior>"
  Bus Selector9/26 -> Mux9/26  "<CAM_TGT_26A_CAN_Tgt_26_Spd_Y>"
  Bus Selector9/27 -> Mux9/27  "<CAM_TGT_27A_CAN_Tgt_27_Spd_Y>"
  Bus Selector15/9 -> Mux15/9  "<CAM_TGT_09B_CAN_Tgt_09_Accel>"
  Bus Selector15/31 -> Mux15/31  "<CAM_TGT_31B_CAN_Tgt_31_Accel>"
  Bus Selector15/19 -> Mux15/19  "<CAM_TGT_19B_CAN_Tgt_19_Accel>"
  Bus Selector9/1 -> Mux9/1  "<CAM_TGT_01A_CAN_Tgt_01_Spd_Y>"
  Bus Selector5/2 -> Mux5/2  "<CAM_TGT_02A_CAN_Tgt_02_Behavior>"
  Bus Selector5/9 -> Mux5/9  "<CAM_TGT_09A_CAN_Tgt_09_Behavior>"
  Bus Selector13/5 -> Mux13/5  "<CAM_TGT_05B_CAN_Tgt_05_Length>"
  Bus Selector5/11 -> Mux5/11  "<CAM_TGT_11A_CAN_Tgt_11_Behavior>"
  Mux1/1 -> Pos_Y_Quality/1
  Bus Selector8/4 -> Mux8/4  "<CAM_TGT_04A_CAN_Tgt_04_Spd_X>"
  Bus Selector5/18 -> Mux5/18  "<CAM_TGT_18A_CAN_Tgt_18_Behavior>"
  Bus Selector5/17 -> Mux5/17  "<CAM_TGT_17A_CAN_Tgt_17_Behavior>"
  Bus Selector5/14 -> Mux5/14  "<CAM_TGT_14A_CAN_Tgt_14_Behavior>"
  Bus Selector5/16 -> Mux5/16  "<CAM_TGT_16A_CAN_Tgt_16_Behavior>"
  Bus Selector15/30 -> Mux15/30  "<CAM_TGT_30B_CAN_Tgt_30_Accel>"
  Bus Selector15/17 -> Mux15/17  "<CAM_TGT_17B_CAN_Tgt_17_Accel>"
  Bus Selector4/27 -> Mux4/27  "<CAM_TGT_27A_CAN_Tgt_27_Pos_X_Quality>"
  Bus Selector7/19 -> Mux7/19  "<CAM_TGT_19A_CAN_Tgt_19_Spd_Y_Quality>"
  Bus Selector15/2 -> Mux15/2  "<CAM_TGT_02B_CAN_Tgt_02_Accel>"
  Bus Selector7/24 -> Mux7/24  "<CAM_TGT_24A_CAN_Tgt_24_Spd_Y_Quality>"
  Bus Selector/3 -> Mux/3  "<CAM_TGT_03A_CAN_Tgt_03_ID>"
  Bus Selector11/8 -> Mux11/8  "<CAM_TGT_08A_CAN_Tgt_08_Pos_X>"
  Bus Selector15/1 -> Mux15/1  "<CAM_TGT_01B_CAN_Tgt_01_Accel>"
  Bus Selector6/14 -> Mux6/14  "<CAM_TGT_14A_CAN_Tgt_14_Stat>"
  Bus Selector/28 -> Mux/28  "<CAM_TGT_28A_CAN_Tgt_28_ID>"
  Bus Selector15/7 -> Mux15/7  "<CAM_TGT_07B_CAN_Tgt_07_Accel>"
  Bus Selector10/11 -> Mux10/11  "<CAM_TGT_11A_CAN_Tgt_11_Pos_Y>"
  Bus Selector10/12 -> Mux10/12  "<CAM_TGT_12A_CAN_Tgt_12_Pos_Y>"
  Bus Selector16/8 -> Mux16/8  "<CAM_TGT_08B_CAN_Tgt_08_Ttc>"
  Bus Selector15/11 -> Mux15/11  "<CAM_TGT_11B_CAN_Tgt_11_Accel>"
  Bus Selector8/31 -> Mux8/31  "<CAM_TGT_31A_CAN_Tgt_31_Spd_X>"
  Bus Selector/19 -> Mux/19  "<CAM_TGT_19A_CAN_Tgt_19_ID>"
  Bus Selector3/21 -> Mux3/21  "<CAM_TGT_21A_CAN_Tgt_21_Spd_X_Quality>"
  Bus Selector16/6 -> Mux16/6  "<CAM_TGT_06B_CAN_Tgt_06_Ttc>"
  Bus Selector15/10 -> Mux15/10  "<CAM_TGT_10B_CAN_Tgt_10_Accel>"
  Bus Selector6/29 -> Mux6/29  "<CAM_TGT_29A_CAN_Tgt_29_Stat>"
  Bus Selector/16 -> Mux/16  "<CAM_TGT_16A_CAN_Tgt_16_ID>"
  Bus Selector16/16 -> Mux16/16  "<CAM_TGT_16B_CAN_Tgt_16_Ttc>"
  Bus Selector15/16 -> Mux15/16  "<CAM_TGT_16B_CAN_Tgt_16_Accel>"
  Bus Selector15/14 -> Mux15/14  "<CAM_TGT_14B_CAN_Tgt_14_Accel>"
  Bus Selector15/21 -> Mux15/21  "<CAM_TGT_21B_CAN_Tgt_21_Accel>"
  Bus Selector15/23 -> Mux15/23  "<CAM_TGT_23B_CAN_Tgt_23_Accel>"
  Bus Selector8/26 -> Mux8/26  "<CAM_TGT_26A_CAN_Tgt_26_Spd_X>"
  Bus Selector4/23 -> Mux4/23  "<CAM_TGT_23A_CAN_Tgt_23_Pos_X_Quality>"
  Bus Selector15/26 -> Mux15/26  "<CAM_TGT_26B_CAN_Tgt_26_Accel>"
  Bus Selector15/24 -> Mux15/24  "<CAM_TGT_24B_CAN_Tgt_24_Accel>"
  Bus Selector15/29 -> Mux15/29  "<CAM_TGT_29B_CAN_Tgt_29_Accel>"
  Bus Selector15/27 -> Mux15/27  "<CAM_TGT_27B_CAN_Tgt_27_Accel>"
  Bus Selector8/32 -> Mux8/32  "<CAM_TGT_32A_CAN_Tgt_32_Spd_X>"
  Bus Selector8/12 -> Mux8/12  "<CAM_TGT_12A_CAN_Tgt_12_Spd_X>"
  Bus Selector8/2 -> Mux8/2  "<CAM_TGT_02A_CAN_Tgt_02_Spd_X>"
  Bus Selector8/3 -> Mux8/3  "<CAM_TGT_03A_CAN_Tgt_03_Spd_X>"
  Bus Selector8/5 -> Mux8/5  "<CAM_TGT_05A_CAN_Tgt_05_Spd_X>"
  Bus Selector4/5 -> Mux4/5  "<CAM_TGT_05A_CAN_Tgt_05_Pos_X_Quality>"
  Bus Selector8/8 -> Mux8/8  "<CAM_TGT_08A_CAN_Tgt_08_Spd_X>"
  Bus Selector8/16 -> Mux8/16  "<CAM_TGT_16A_CAN_Tgt_16_Spd_X>"
  Bus Selector8/14 -> Mux8/14  "<CAM_TGT_14A_CAN_Tgt_14_Spd_X>"
  Bus Selector16/10 -> Mux16/10  "<CAM_TGT_10B_CAN_Tgt_10_Ttc>"
  Bus Selector8/17 -> Mux8/17  "<CAM_TGT_17A_CAN_Tgt_17_Spd_X>"
  Bus Selector8/19 -> Mux8/19  "<CAM_TGT_19A_CAN_Tgt_19_Spd_X>"
  Bus Selector8/27 -> Mux8/27  "<CAM_TGT_27A_CAN_Tgt_27_Spd_X>"
  Bus Selector8/22 -> Mux8/22  "<CAM_TGT_22A_CAN_Tgt_22_Spd_X>"
  Bus Selector8/29 -> Mux8/29  "<CAM_TGT_29A_CAN_Tgt_29_Spd_X>"
  Bus Selector13/16 -> Mux13/16  "<CAM_TGT_16B_CAN_Tgt_16_Length>"
  Bus Selector3/19 -> Mux3/19  "<CAM_TGT_19A_CAN_Tgt_19_Spd_X_Quality>"
  Bus Selector4/3 -> Mux4/3  "<CAM_TGT_03A_CAN_Tgt_03_Pos_X_Quality>"
  Bus Selector13/24 -> Mux13/24  "<CAM_TGT_24B_CAN_Tgt_24_Length>"
  Bus Selector10/13 -> Mux10/13  "<CAM_TGT_13A_CAN_Tgt_13_Pos_Y>"
  Bus Selector4/7 -> Mux4/7  "<CAM_TGT_07A_CAN_Tgt_07_Pos_X_Quality>"
  Bus Selector4/10 -> Mux4/10  "<CAM_TGT_10A_CAN_Tgt_10_Pos_X_Quality>"
  Bus Selector4/11 -> Mux4/11  "<CAM_TGT_11A_CAN_Tgt_11_Pos_X_Quality>"
  Bus Selector4/19 -> Mux4/19  "<CAM_TGT_19A_CAN_Tgt_19_Pos_X_Quality>"
  Bus Selector11/12 -> Mux11/12  "<CAM_TGT_12A_CAN_Tgt_12_Pos_X>"
  Bus Selector11/4 -> Mux11/4  "<CAM_TGT_04A_CAN_Tgt_04_Pos_X>"
  Bus Selector16/17 -> Mux16/17  "<CAM_TGT_17B_CAN_Tgt_17_Ttc>"
  Bus Selector4/14 -> Mux4/14  "<CAM_TGT_14A_CAN_Tgt_14_Pos_X_Quality>"
  Mux13/1 -> Length/1
  Bus Selector11/15 -> Mux11/15  "<CAM_TGT_15A_CAN_Tgt_15_Pos_X>"
  Bus Selector3/2 -> Mux3/2  "<CAM_TGT_02A_CAN_Tgt_02_Spd_X_Quality>"
  Bus Selector7/9 -> Mux7/9  "<CAM_TGT_09A_CAN_Tgt_09_Spd_Y_Quality>"
  Bus Selector4/24 -> Mux4/24  "<CAM_TGT_24A_CAN_Tgt_24_Pos_X_Quality>"
  Bus Selector4/28 -> Mux4/28  "<CAM_TGT_28A_CAN_Tgt_28_Pos_X_Quality>"
  Bus Selector10/27 -> Mux10/27  "<CAM_TGT_27A_CAN_Tgt_27_Pos_Y>"
  Bus Selector10/2 -> Mux10/2  "<CAM_TGT_02A_CAN_Tgt_02_Pos_Y>"
  Bus Selector10/6 -> Mux10/6  "<CAM_TGT_06A_CAN_Tgt_06_Pos_Y>"
  Bus Selector13/26 -> Mux13/26  "<CAM_TGT_26B_CAN_Tgt_26_Length>"
  Bus Selector10/20 -> Mux10/20  "<CAM_TGT_20A_CAN_Tgt_20_Pos_Y>"
  Bus Selector10/21 -> Mux10/21  "<CAM_TGT_21A_CAN_Tgt_21_Pos_Y>"
  Bus Selector11/6 -> Mux11/6  "<CAM_TGT_06A_CAN_Tgt_06_Pos_X>"
  Bus Selector10/25 -> Mux10/25  "<CAM_TGT_25A_CAN_Tgt_25_Pos_Y>"
  Bus Selector10/22 -> Mux10/22  "<CAM_TGT_22A_CAN_Tgt_22_Pos_Y>"
  Bus Selector16/7 -> Mux16/7  "<CAM_TGT_07B_CAN_Tgt_07_Ttc>"
  Bus Selector10/28 -> Mux10/28  "<CAM_TGT_28A_CAN_Tgt_28_Pos_Y>"
  Bus Selector7/11 -> Mux7/11  "<CAM_TGT_11A_CAN_Tgt_11_Spd_Y_Quality>"
  Bus Selector11/29 -> Mux11/29  "<CAM_TGT_29A_CAN_Tgt_29_Pos_X>"
  Bus Selector10/31 -> Mux10/31  "<CAM_TGT_31A_CAN_Tgt_31_Pos_Y>"
  Bus Selector7/5 -> Mux7/5  "<CAM_TGT_05A_CAN_Tgt_05_Spd_Y_Quality>"
  Bus Selector11/32 -> Mux11/32  "<CAM_TGT_32A_CAN_Tgt_32_Pos_X>"
  Bus Selector11/2 -> Mux11/2  "<CAM_TGT_02A_CAN_Tgt_02_Pos_X>"
  Mux8/1 -> Spd_X/1
  Bus Selector11/3 -> Mux11/3  "<CAM_TGT_03A_CAN_Tgt_03_Pos_X>"
  Bus Selector11/7 -> Mux11/7  "<CAM_TGT_07A_CAN_Tgt_07_Pos_X>"
  Bus Selector11/17 -> Mux11/17  "<CAM_TGT_17A_CAN_Tgt_17_Pos_X>"
  Bus Selector11/14 -> Mux11/14  "<CAM_TGT_14A_CAN_Tgt_14_Pos_X>"
  Bus Selector11/24 -> Mux11/24  "<CAM_TGT_24A_CAN_Tgt_24_Pos_X>"
  Bus Selector11/23 -> Mux11/23  "<CAM_TGT_23A_CAN_Tgt_23_Pos_X>"
  Bus Selector13/9 -> Mux13/9  "<CAM_TGT_09B_CAN_Tgt_09_Length>"
  Bus Selector11/30 -> Mux11/30  "<CAM_TGT_30A_CAN_Tgt_30_Pos_X>"
  Bus Selector16/15 -> Mux16/15  "<CAM_TGT_15B_CAN_Tgt_15_Ttc>"
  Bus Selector6/15 -> Mux6/15  "<CAM_TGT_15A_CAN_Tgt_15_Stat>"
  Bus Selector16/24 -> Mux16/24  "<CAM_TGT_24B_CAN_Tgt_24_Ttc>"
  Bus Selector16/1 -> Mux16/1  "<CAM_TGT_01B_CAN_Tgt_01_Ttc>"
  Bus Selector16/13 -> Mux16/13  "<CAM_TGT_13B_CAN_Tgt_13_Ttc>"
  Bus Selector3/1 -> Mux3/1  "<CAM_TGT_01A_CAN_Tgt_01_Spd_X_Quality>"
  Bus Selector16/12 -> Mux16/12  "<CAM_TGT_12B_CAN_Tgt_12_Ttc>"
  Bus Selector/20 -> Mux/20  "<CAM_TGT_20A_CAN_Tgt_20_ID>"
  Bus Selector/17 -> Mux/17  "<CAM_TGT_17A_CAN_Tgt_17_ID>"
  Bus Selector/23 -> Mux/23  "<CAM_TGT_23A_CAN_Tgt_23_ID>"
  Bus Selector/24 -> Mux/24  "<CAM_TGT_24A_CAN_Tgt_24_ID>"
  Bus Selector/30 -> Mux/30  "<CAM_TGT_30A_CAN_Tgt_30_ID>"
  Bus Selector/27 -> Mux/27  "<CAM_TGT_27A_CAN_Tgt_27_ID>"
  Bus Selector3/3 -> Mux3/3  "<CAM_TGT_03A_CAN_Tgt_03_Spd_X_Quality>"
  Bus Selector/11 -> Mux/11  "<CAM_TGT_11A_CAN_Tgt_11_ID>"
  Bus Selector7/1 -> Mux7/1  "<CAM_TGT_01A_CAN_Tgt_01_Spd_Y_Quality>"
  Bus Selector7/2 -> Mux7/2  "<CAM_TGT_02A_CAN_Tgt_02_Spd_Y_Quality>"
  Bus Selector3/5 -> Mux3/5  "<CAM_TGT_05A_CAN_Tgt_05_Spd_X_Quality>"
  Bus Selector7/8 -> Mux7/8  "<CAM_TGT_08A_CAN_Tgt_08_Spd_Y_Quality>"
  Bus Selector7/16 -> Mux7/16  "<CAM_TGT_16A_CAN_Tgt_16_Spd_Y_Quality>"
  Bus Selector13/1 -> Mux13/1  "<CAM_TGT_01B_CAN_Tgt_01_Length>"
  Bus Selector7/26 -> Mux7/26  "<CAM_TGT_26A_CAN_Tgt_26_Spd_Y_Quality>"
  Bus Selector7/29 -> Mux7/29  "<CAM_TGT_29A_CAN_Tgt_29_Spd_Y_Quality>"
  Bus Selector13/3 -> Mux13/3  "<CAM_TGT_03B_CAN_Tgt_03_Length>"
  Bus Selector13/6 -> Mux13/6  "<CAM_TGT_06B_CAN_Tgt_06_Length>"
  Bus Selector13/7 -> Mux13/7  "<CAM_TGT_07B_CAN_Tgt_07_Length>"
  Bus Selector13/10 -> Mux13/10  "<CAM_TGT_10B_CAN_Tgt_10_Length>"
  Bus Selector13/15 -> Mux13/15  "<CAM_TGT_15B_CAN_Tgt_15_Length>"
  Bus Selector13/18 -> Mux13/18  "<CAM_TGT_18B_CAN_Tgt_18_Length>"
  Bus Selector13/19 -> Mux13/19  "<CAM_TGT_19B_CAN_Tgt_19_Length>"
  Bus Selector3/10 -> Mux3/10  "<CAM_TGT_10A_CAN_Tgt_10_Spd_X_Quality>"
  Bus Selector13/17 -> Mux13/17  "<CAM_TGT_17B_CAN_Tgt_17_Length>"
  Bus Selector13/20 -> Mux13/20  "<CAM_TGT_20B_CAN_Tgt_20_Length>"
  Bus Selector13/23 -> Mux13/23  "<CAM_TGT_23B_CAN_Tgt_23_Length>"
  Bus Selector3/6 -> Mux3/6  "<CAM_TGT_06A_CAN_Tgt_06_Spd_X_Quality>"
  Bus Selector3/7 -> Mux3/7  "<CAM_TGT_07A_CAN_Tgt_07_Spd_X_Quality>"
  Bus Selector3/11 -> Mux3/11  "<CAM_TGT_11A_CAN_Tgt_11_Spd_X_Quality>"
  Bus Selector3/14 -> Mux3/14  "<CAM_TGT_14A_CAN_Tgt_14_Spd_X_Quality>"
  Bus Selector3/17 -> Mux3/17  "<CAM_TGT_17A_CAN_Tgt_17_Spd_X_Quality>"
  Bus Selector3/26 -> Mux3/26  "<CAM_TGT_26A_CAN_Tgt_26_Spd_X_Quality>"
  Bus Selector3/25 -> Mux3/25  "<CAM_TGT_25A_CAN_Tgt_25_Spd_X_Quality>"
  Bus Selector3/28 -> Mux3/28  "<CAM_TGT_28A_CAN_Tgt_28_Spd_X_Quality>"
  Bus Selector3/27 -> Mux3/27  "<CAM_TGT_27A_CAN_Tgt_27_Spd_X_Quality>"
  Bus Selector3/30 -> Mux3/30  "<CAM_TGT_30A_CAN_Tgt_30_Spd_X_Quality>"
  Bus Selector3/31 -> Mux3/31  "<CAM_TGT_31A_CAN_Tgt_31_Spd_X_Quality>"
  Bus Selector6/1 -> Mux6/1  "<CAM_TGT_01A_CAN_Tgt_01_Stat>"
  Bus Selector6/2 -> Mux6/2  "<CAM_TGT_02A_CAN_Tgt_02_Stat>"
  Bus Selector6/11 -> Mux6/11  "<CAM_TGT_11A_CAN_Tgt_11_Stat>"
  Bus Selector6/13 -> Mux6/13  "<CAM_TGT_13A_CAN_Tgt_13_Stat>"
  Bus Selector6/18 -> Mux6/18  "<CAM_TGT_18A_CAN_Tgt_18_Stat>"
  Bus Selector6/24 -> Mux6/24  "<CAM_TGT_24A_CAN_Tgt_24_Stat>"
  Bus Selector6/22 -> Mux6/22  "<CAM_TGT_22A_CAN_Tgt_22_Stat>"
  Bus Selector6/31 -> Mux6/31  "<CAM_TGT_31A_CAN_Tgt_31_Stat>"
  Bus Selector6/28 -> Mux6/28  "<CAM_TGT_28A_CAN_Tgt_28_Stat>"
  Mux/1 -> ID/1

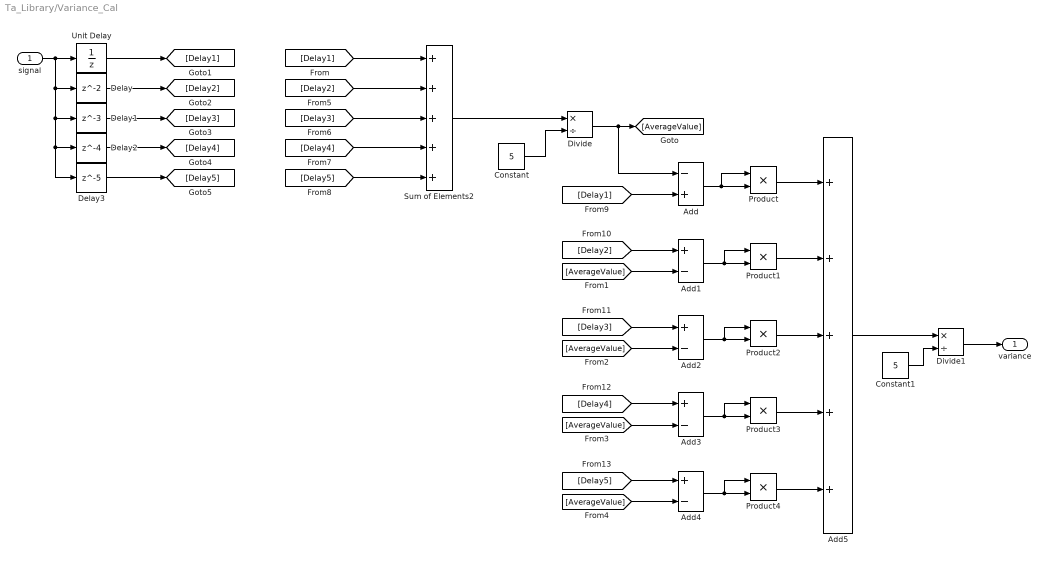
== system Ta_Library/Variance_Cal ==
  signal : Inport
  Add : Sum  Inputs=-+
  Add{1..4} (4 alike) : Sum  Inputs=+-
  Add5 : Sum  Inputs=+++++
  Constant : Constant  Value=5  OutDataTypeStr=single
  Constant1 : Constant  Value=5  OutDataTypeStr=single
  Delay : Delay
  Delay1 : Delay  DelayLength=3
  Delay2 : Delay  DelayLength=4
  Delay3 : Delay  DelayLength=5
  Divide : Product  Inputs=*/
  Divide1 : Product  Inputs=*/
  Product{,1..4} (5 alike) : Product
  Sum of Elements2 : Sum  Inputs=+++++
  Unit Delay : UnitDelay  SampleTime=-1  HasFrameUpgradeWarning=on
  variance : Outport
  wires:
  Constant/1 -> Divide/2
  Divide/1 -> Add/1, [AverageValue]
  Add/1 -> Product/1, Product/2
  [AverageValue] -> Add1/2
  Add1/1 -> Product1/1, Product1/2
  Add2/1 -> Product2/1, Product2/2
  [AverageValue] -> Add2/2
  [AverageValue] -> Add3/2
  Add3/1 -> Product3/1, Product3/2
  Add4/1 -> Product4/1, Product4/2
  [AverageValue] -> Add4/2
  Product/1 -> Add5/1
  Product1/1 -> Add5/2
  Product2/1 -> Add5/3
  Product3/1 -> Add5/4
  Product4/1 -> Add5/5
  Add5/1 -> Divide1/1
  Constant1/1 -> Divide1/2
  Divide1/1 -> variance/1
  [Delay1] -> Sum of Elements2/1
  [Delay2] -> Sum of Elements2/2
  [Delay3] -> Sum of Elements2/3
  [Delay4] -> Sum of Elements2/4
  [Delay5] -> Sum of Elements2/5
  Sum of Elements2/1 -> Divide/1
  [Delay5] -> Add4/1
  [Delay4] -> Add3/1
  [Delay3] -> Add2/1
  [Delay2] -> Add1/1
  [Delay1] -> Add/2
  signal/1 -> Delay3/1, Delay2/1, Delay1/1, Delay/1, Unit Delay/1
  Unit Delay/1 -> [Delay1]
  Delay/1 -> [Delay2]
  Delay1/1 -> [Delay3]
  Delay2/1 -> [Delay4]
  Delay3/1 -> [Delay5]
